simulink model "ConSys_A1"  (Simulink 8.3)
settings: Solver=ode3  StartTime=0.0  StopTime=Time(end)  FixedStep=Ts  RelTol=1e-3
values from neighbouring files (symbols this model uses):
  d = r*h    (= 1.6)    [StartUp_A1.m]
  d0 = d*h    (= 0.0032)    [StartUp_A1.m]
  h = 0.002    [StartUp_A1.m]
  Ka = diag([ 3  20  20  150  355  520])    [StartUp_A1.m]
  Kd = diag([ 3   5  25  100   15 1050])    [StartUp_A1.m]
  Ki = diag([35 555 810 7410 1850 5815])    [StartUp_A1.m]
  Kp = diag([55 180 350 1960  680 4450])    [StartUp_A1.m]
  r = 800    [StartUp_A1.m]
  TD = ss(Atd,Btd,Ctd,Dtd,Ts)    [StartUp_A1.m]
  Ts = 1/200    (= 0.005)    [StartUp_A1.m]
undefined symbols (not defined in the file or in its folder): DiscIntNeverNeededParam
undefined symbols (not defined in the file): ADAMS_cwd, ADAMS_exec, ADAMS_host, ADAMS_init, ADAMS_inputs, ADAMS_outputs, ADAMS_prefix, ADAMS_static, ADAMS_sysdir
libraries: cstblocks x6
(part 7 of 9)

== matlab function A2/MATLAB Function 4 ==
  data: q input double; V4 output double; dq input double
function V4 = V4(q,dq)
%#codegen
Th1=q(1,1); Th2=q(2,1); Th3=q(3,1); Th4=q(4,1); Th5=q(5,1); Th6=q(6,1);
dTh1=dq(1); dTh2=dq(2); dTh3=dq(3); dTh4=dq(4); dTh5=dq(5); dTh6=dq(6);
%---------------------------
V411=((0.000115*cos(Th4)*sin(Th6) - 0.02603*sin(Th4)*sin(Th5) + 0.000115*cos(Th5)*cos(Th6)*sin(Th4))*(0.07*sin(Th2 + Th3) + 0.063*sin(2.0*Th2 + 2.0*Th3) - 0.36*sin(Th2 + Th3)*sin(Th2) + 0.05206*cos(Th4)*sin(Th5) + 0.00023*sin(Th4)*sin(Th6) + 0.254*sin(Th2 + Th3)*cos(Th2)*cos(Th3) - 0.254*sin(Th2 + Th3)*sin(Th2)*sin(Th3) - 0.00023*cos(Th4)*cos(Th5)*cos(Th6) - 0.05206*sin(Th2 + Th3)^2*cos(Th4)*sin(Th5) - 0.00023*sin(Th2 + Th3)^2*sin(Th4)*sin(Th6) + 0.05206*cos(Th2 + Th3)*sin(Th2 + Th3)*cos(Th5) + 0.00023*sin(Th2 + Th3)^2*cos(Th4)*cos(Th5)*cos(Th6) + 0.00023*cos(Th2 + Th3)*sin(Th2 + Th3)*cos(Th6)*sin(Th5)) - 1.0*(0.00062*cos(Th4) - 0.00002*cos(Th5)*sin(Th4) + 0.00152*sin(Th4)*sin(Th5))*(0.00062*sin(Th2 + Th3)^2*sin(Th4) - 0.063*sin(2.0*Th2 + 2.0*Th3) - 0.00062*sin(Th4) - 0.07*sin(Th2 + Th3) + 0.36*sin(Th2 + Th3)*sin(Th2) - 0.00002*cos(Th4)*cos(Th5) + 0.00152*cos(Th4)*sin(Th5) + 0.00002*cos(Th2 + Th3)*sin(Th2 + Th3)*sin(Th5) - 0.254*sin(Th2 + Th3)*cos(Th2)*cos(Th3) + 0.254*sin(Th2 + Th3)*sin(Th2)*sin(Th3) + 0.00002*sin(Th2 + Th3)^2*cos(Th4)*cos(Th5) - 0.00152*sin(Th2 + Th3)^2*cos(Th4)*sin(Th5) + 0.00152*cos(Th2 + Th3)*sin(Th2 + Th3)*cos(Th5)) - 1.1369e-18*cos(Th2 + Th3)*(3.5184e13*cos(Th2 + Th3)*sin(Th5) + 4.1368e15*cos(Th2 + Th3)*cos(Th4)*sin(Th4) - 3.5184e13*sin(Th2 + Th3)*cos(Th4)*cos(Th5) - 7.0369e13*cos(Th2 + Th3)*cos(Th4)^2*sin(Th5) + 3.8782e15*sin(Th2 + Th3)*cos(Th5)*sin(Th4)*sin(Th5) - 3.8782e15*cos(Th2 + Th3)*cos(Th4)*cos(Th5)^2*sin(Th4)) - 4.2352e-22*cos(Th2 + Th3)*(1.2314e18*cos(Th4)*sin(Th6) + 4.7224e15*sin(Th4)*sin(Th5) + 1.2314e18*cos(Th5)*cos(Th6)*sin(Th4))*(cos(Th2 + Th3)*sin(Th4)*sin(Th6) + sin(Th2 + Th3)*cos(Th6)*sin(Th5) - 1.0*cos(Th2 + Th3)*cos(Th4)*cos(Th5)*cos(Th6)) - 0.00052*cos(Th2 + Th3)*(cos(Th4)*cos(Th6) - 1.0*cos(Th5)*sin(Th4)*sin(Th6))*(cos(Th2 + Th3)*cos(Th6)*sin(Th4) - 1.0*sin(Th2 + Th3)*sin(Th5)*sin(Th6) + cos(Th2 + Th3)*cos(Th4)*cos(Th5)*sin(Th6)) - 0.004593*cos(Th2 + Th3)^2*cos(Th4)*sin(Th4) - 0.5*cos(Th2 + Th3)*(cos(Th4)*cos(Th6) - 1.0*cos(Th5)*sin(Th4)*sin(Th6))*(0.00104*cos(Th2 + Th3)*cos(Th6)*sin(Th4) - 0.00104*sin(Th2 + Th3)*sin(Th5)*sin(Th6) + 0.00104*cos(Th2 + Th3)*cos(Th4)*cos(Th5)*sin(Th6)) + 0.5*cos(Th2 + Th3)*(cos(Th4)*sin(Th6) + cos(Th5)*cos(Th6)*sin(Th4))*(4.0e-6*sin(Th2 + Th3)*cos(Th5) + 4.0e-6*cos(Th2 + Th3)*cos(Th4)*sin(Th5) - 0.001043*cos(Th2 + Th3)*sin(Th4)*sin(Th6) - 0.001043*sin(Th2 + Th3)*cos(Th6)*sin(Th5) + 0.001043*cos(Th2 + Th3)*cos(Th4)*cos(Th5)*cos(Th6)) + 4.2352e-22*cos(Th2 + Th3)*(sin(Th2 + Th3)*cos(Th5) + cos(Th2 + Th3)*cos(Th4)*sin(Th5))*(4.7224e15*cos(Th4)*sin(Th6) + 1.3695e17*sin(Th4)*sin(Th5) + 4.7224e15*cos(Th5)*cos(Th6)*sin(Th4)) + 0.5*cos(Th2 + Th3)*sin(Th4)*sin(Th5)*(0.000116*sin(Th2 + Th3)*cos(Th5) + 0.000116*cos(Th2 + Th3)*cos(Th4)*sin(Th5) - 4.0e-6*cos(Th2 + Th3)*sin(Th4)*sin(Th6) - 4.0e-6*sin(Th2 + Th3)*cos(Th6)*sin(Th5) + 4.0e-6*cos(Th2 + Th3)*cos(Th4)*cos(Th5)*cos(Th6)))*dTh1*dTh1;
V412=(0.0064488*cos(Th2)*cos(Th3) + 0.0003348*cos(Th2)*sin(Th4) - 0.0064488*sin(Th2)*sin(Th3) - 0.01158*cos(Th4)^2*sin(Th2)*sin(Th3) + 0.0033452*cos(Th5)^2*sin(Th2)*sin(Th3) - 4.4603e-6*cos(Th6)^2*sin(Th2)*sin(Th3) + 0.0000108*cos(Th2)*cos(Th4)*cos(Th5) + 4.56e-8*cos(Th2)*cos(Th4)*sin(Th3) + 4.56e-8*cos(Th3)*cos(Th4)*sin(Th2) + 0.013235*cos(Th2)*cos(Th4)*sin(Th5) + 0.0003534*cos(Th2)*sin(Th3)*sin(Th4) + 0.0003534*cos(Th3)*sin(Th2)*sin(Th4) + 0.0000621*cos(Th2)*sin(Th4)*sin(Th6) + 0.01158*cos(Th2)*cos(Th3)*cos(Th4)^2 - 0.0033452*cos(Th2)*cos(Th3)*cos(Th5)^2 + 4.4603e-6*cos(Th2)*cos(Th3)*cos(Th6)^2 + 0.0066904*cos(Th4)^2*cos(Th5)^2*sin(Th2)*sin(Th3) + 2.9736e-6*cos(Th4)^2*cos(Th6)^2*sin(Th2)*sin(Th3) + 1.4868e-6*cos(Th5)^2*cos(Th6)^2*sin(Th2)*sin(Th3) - 0.0000621*cos(Th2)*cos(Th4)*cos(Th5)*cos(Th6) + 0.0000114*cos(Th2)*cos(Th4)*cos(Th5)*sin(Th3) + 0.0000114*cos(Th3)*cos(Th4)*cos(Th5)*sin(Th2) - 3.04e-8*cos(Th2)*cos(Th3)*cos(Th5)*sin(Th5) + 0.00001498*cos(Th2)*cos(Th4)*cos(Th6)*sin(Th3) + 0.00001498*cos(Th3)*cos(Th4)*cos(Th6)*sin(Th2) + 0.013971*cos(Th2)*cos(Th4)*sin(Th3)*sin(Th5) + 0.000058586*cos(Th2)*cos(Th5)*sin(Th3)*sin(Th4) + 0.013971*cos(Th3)*cos(Th4)*sin(Th2)*sin(Th5) + 0.000058586*cos(Th3)*cos(Th5)*sin(Th2)*sin(Th4) - 1.86e-8*cos(Th2)*sin(Th3)*sin(Th4)*sin(Th5) - 1.86e-8*cos(Th3)*sin(Th2)*sin(Th4)*sin(Th5) + 0.00006555*cos(Th2)*sin(Th3)*sin(Th4)*sin(Th6) + 0.00006555*cos(Th3)*sin(Th2)*sin(Th4)*sin(Th6) + 3.04e-8*cos(Th5)*sin(Th2)*sin(Th3)*sin(Th5) - 9.12e-8*cos(Th2)*cos(Th4)*cos(Th5)^2*sin(Th3) - 9.12e-8*cos(Th3)*cos(Th4)*cos(Th5)^2*sin(Th2) - 0.0066904*cos(Th2)*cos(Th3)*cos(Th4)^2*cos(Th5)^2 - 2.9736e-6*cos(Th2)*cos(Th3)*cos(Th4)^2*cos(Th6)^2 - 1.4868e-6*cos(Th2)*cos(Th3)*cos(Th5)^2*cos(Th6)^2 + 2.48e-8*cos(Th2)*cos(Th3)*cos(Th4)*cos(Th5)*sin(Th4) - 0.00006555*cos(Th2)*cos(Th4)*cos(Th5)*cos(Th6)*sin(Th3) - 0.00006555*cos(Th3)*cos(Th4)*cos(Th5)*cos(Th6)*sin(Th2) - 9.9869e-6*cos(Th2)*cos(Th3)*cos(Th5)*cos(Th6)*sin(Th5) - 2.9736e-6*cos(Th2)*cos(Th3)*cos(Th4)^2*cos(Th5)^2*cos(Th6)^2 + 0.000078115*cos(Th2)*cos(Th3)*cos(Th4)*sin(Th4)*sin(Th5) + 0.010036*cos(Th2)*cos(Th4)*cos(Th5)*sin(Th3)*sin(Th5) + 0.010036*cos(Th3)*cos(Th4)*cos(Th5)*sin(Th2)*sin(Th5) - 2.48e-8*cos(Th4)*cos(Th5)*sin(Th2)*sin(Th3)*sin(Th4) + 0.00001498*cos(Th2)*cos(Th5)*sin(Th3)*sin(Th4)*sin(Th6) + 0.00001498*cos(Th3)*cos(Th5)*sin(Th2)*sin(Th4)*sin(Th6) + 9.9869e-6*cos(Th5)*cos(Th6)*sin(Th2)*sin(Th3)*sin(Th5) + 2.9736e-6*cos(Th4)^2*cos(Th5)^2*cos(Th6)^2*sin(Th2)*sin(Th3) - 0.000078115*cos(Th4)*sin(Th2)*sin(Th3)*sin(Th4)*sin(Th5) - 6.08e-8*cos(Th2)*cos(Th3)*cos(Th4)^2*cos(Th5)*sin(Th5) - 0.000029961*cos(Th2)*cos(Th4)*cos(Th5)^2*cos(Th6)*sin(Th3) - 0.000029961*cos(Th3)*cos(Th4)*cos(Th5)^2*cos(Th6)*sin(Th2) + 6.08e-8*cos(Th4)^2*cos(Th5)*sin(Th2)*sin(Th3)*sin(Th5) - 0.000019974*cos(Th2)*cos(Th3)*cos(Th4)^2*cos(Th5)*cos(Th6)*sin(Th5) + 4.4603e-6*cos(Th2)*cos(Th4)*cos(Th5)*cos(Th6)^2*sin(Th3)*sin(Th5) + 4.4603e-6*cos(Th3)*cos(Th4)*cos(Th5)*cos(Th6)^2*sin(Th2)*sin(Th5) + 0.000019974*cos(Th4)^2*cos(Th5)*cos(Th6)*sin(Th2)*sin(Th3)*sin(Th5) + 0.000019974*cos(Th2)*cos(Th3)*cos(Th4)*sin(Th4)*sin(Th5)*sin(Th6) - 4.4603e-6*cos(Th2)*cos(Th6)*sin(Th3)*sin(Th4)*sin(Th5)*sin(Th6) - 4.4603e-6*cos(Th3)*cos(Th6)*sin(Th2)*sin(Th4)*sin(Th5)*sin(Th6) - 0.000019974*cos(Th4)*sin(Th2)*sin(Th3)*sin(Th4)*sin(Th5)*sin(Th6) + 5.9471e-6*cos(Th2)*cos(Th3)*cos(Th4)*cos(Th5)*cos(Th6)*sin(Th4)*sin(Th6) - 5.9471e-6*cos(Th4)*cos(Th5)*cos(Th6)*sin(Th2)*sin(Th3)*sin(Th4)*sin(Th6))*dTh1*dTh2;
V413=(0.0064488*cos(Th2)*cos(Th3) - 0.0064488*sin(Th2)*sin(Th3) - 0.01158*cos(Th4)^2*sin(Th2)*sin(Th3) + 0.0033452*cos(Th5)^2*sin(Th2)*sin(Th3) - 4.4603e-6*cos(Th6)^2*sin(Th2)*sin(Th3) + 4.56e-8*cos(Th2)*cos(Th4)*sin(Th3) + 4.56e-8*cos(Th3)*cos(Th4)*sin(Th2) + 0.0003534*cos(Th2)*sin(Th3)*sin(Th4) + 0.0003534*cos(Th3)*sin(Th2)*sin(Th4) + 0.01158*cos(Th2)*cos(Th3)*cos(Th4)^2 - 0.0033452*cos(Th2)*cos(Th3)*cos(Th5)^2 + 4.4603e-6*cos(Th2)*cos(Th3)*cos(Th6)^2 + 0.0066904*cos(Th4)^2*cos(Th5)^2*sin(Th2)*sin(Th3) + 2.9736e-6*cos(Th4)^2*cos(Th6)^2*sin(Th2)*sin(Th3) + 1.4868e-6*cos(Th5)^2*cos(Th6)^2*sin(Th2)*sin(Th3) + 0.0000114*cos(Th2)*cos(Th4)*cos(Th5)*sin(Th3) + 0.0000114*cos(Th3)*cos(Th4)*cos(Th5)*sin(Th2) - 3.04e-8*cos(Th2)*cos(Th3)*cos(Th5)*sin(Th5) + 0.00001498*cos(Th2)*cos(Th4)*cos(Th6)*sin(Th3) + 0.00001498*cos(Th3)*cos(Th4)*cos(Th6)*sin(Th2) + 0.013971*cos(Th2)*cos(Th4)*sin(Th3)*sin(Th5) + 0.000058586*cos(Th2)*cos(Th5)*sin(Th3)*sin(Th4) + 0.013971*cos(Th3)*cos(Th4)*sin(Th2)*sin(Th5) + 0.000058586*cos(Th3)*cos(Th5)*sin(Th2)*sin(Th4) - 1.86e-8*cos(Th2)*sin(Th3)*sin(Th4)*sin(Th5) - 1.86e-8*cos(Th3)*sin(Th2)*sin(Th4)*sin(Th5) + 0.00006555*cos(Th2)*sin(Th3)*sin(Th4)*sin(Th6) + 0.00006555*cos(Th3)*sin(Th2)*sin(Th4)*sin(Th6) + 3.04e-8*cos(Th5)*sin(Th2)*sin(Th3)*sin(Th5) - 9.12e-8*cos(Th2)*cos(Th4)*cos(Th5)^2*sin(Th3) - 9.12e-8*cos(Th3)*cos(Th4)*cos(Th5)^2*sin(Th2) - 0.0066904*cos(Th2)*cos(Th3)*cos(Th4)^2*cos(Th5)^2 - 2.9736e-6*cos(Th2)*cos(Th3)*cos(Th4)^2*cos(Th6)^2 - 1.4868e-6*cos(Th2)*cos(Th3)*cos(Th5)^2*cos(Th6)^2 + 2.48e-8*cos(Th2)*cos(Th3)*cos(Th4)*cos(Th5)*sin(Th4) - 0.00006555*cos(Th2)*cos(Th4)*cos(Th5)*cos(Th6)*sin(Th3) - 0.00006555*cos(Th3)*cos(Th4)*cos(Th5)*cos(Th6)*sin(Th2) - 9.9869e-6*cos(Th2)*cos(Th3)*cos(Th5)*cos(Th6)*sin(Th5) - 2.9736e-6*cos(Th2)*cos(Th3)*cos(Th4)^2*cos(Th5)^2*cos(Th6)^2 + 0.000078115*cos(Th2)*cos(Th3)*cos(Th4)*sin(Th4)*sin(Th5) + 0.010036*cos(Th2)*cos(Th4)*cos(Th5)*sin(Th3)*sin(Th5) + 0.010036*cos(Th3)*cos(Th4)*cos(Th5)*sin(Th2)*sin(Th5) - 2.48e-8*cos(Th4)*cos(Th5)*sin(Th2)*sin(Th3)*sin(Th4) + 0.00001498*cos(Th2)*cos(Th5)*sin(Th3)*sin(Th4)*sin(Th6) + 0.00001498*cos(Th3)*cos(Th5)*sin(Th2)*sin(Th4)*sin(Th6) + 9.9869e-6*cos(Th5)*cos(Th6)*sin(Th2)*sin(Th3)*sin(Th5) + 2.9736e-6*cos(Th4)^2*cos(Th5)^2*cos(Th6)^2*sin(Th2)*sin(Th3) - 0.000078115*cos(Th4)*sin(Th2)*sin(Th3)*sin(Th4)*sin(Th5) - 6.08e-8*cos(Th2)*cos(Th3)*cos(Th4)^2*cos(Th5)*sin(Th5) - 0.000029961*cos(Th2)*cos(Th4)*cos(Th5)^2*cos(Th6)*sin(Th3) - 0.000029961*cos(Th3)*cos(Th4)*cos(Th5)^2*cos(Th6)*sin(Th2) + 6.08e-8*cos(Th4)^2*cos(Th5)*sin(Th2)*sin(Th3)*sin(Th5) - 0.000019974*cos(Th2)*cos(Th3)*cos(Th4)^2*cos(Th5)*cos(Th6)*sin(Th5) + 4.4603e-6*cos(Th2)*cos(Th4)*cos(Th5)*cos(Th6)^2*sin(Th3)*sin(Th5) + 4.4603e-6*cos(Th3)*cos(Th4)*cos(Th5)*cos(Th6)^2*sin(Th2)*sin(Th5) + 0.000019974*cos(Th4)^2*cos(Th5)*cos(Th6)*sin(Th2)*sin(Th3)*sin(Th5) + 0.000019974*cos(Th2)*cos(Th3)*cos(Th4)*sin(Th4)*sin(Th5)*sin(Th6) - 4.4603e-6*cos(Th2)*cos(Th6)*sin(Th3)*sin(Th4)*sin(Th5)*sin(Th6) - 4.4603e-6*cos(Th3)*cos(Th6)*sin(Th2)*sin(Th4)*sin(Th5)*sin(Th6) - 0.000019974*cos(Th4)*sin(Th2)*sin(Th3)*sin(Th4)*sin(Th5)*sin(Th6) + 5.9471e-6*cos(Th2)*cos(Th3)*cos(Th4)*cos(Th5)*cos(Th6)*sin(Th4)*sin(Th6) - 5.9471e-6*cos(Th4)*cos(Th5)*cos(Th6)*sin(Th2)*sin(Th3)*sin(Th4)*sin(Th6))*dTh1*dTh3;
V414=(0.0001116*cos(Th4)*sin(Th2) - 0.0000217*cos(Th4) + 7.0e-7*cos(Th5)*sin(Th4) - 4.025e-6*cos(Th4)*sin(Th6) + 0.00085785*sin(Th4)*sin(Th5) - 0.0001178*cos(Th2)*cos(Th3)*cos(Th4) + 1.52e-8*cos(Th2)*cos(Th3)*sin(Th4) - 4.025e-6*cos(Th5)*cos(Th6)*sin(Th4) + 0.0001178*cos(Th4)*sin(Th2)*sin(Th3) - 3.6e-6*cos(Th5)*sin(Th2)*sin(Th4) + 0.0000207*cos(Th4)*sin(Th2)*sin(Th6) - 1.52e-8*sin(Th2)*sin(Th3)*sin(Th4) - 0.0044118*sin(Th2)*sin(Th4)*sin(Th5) - 0.000019529*cos(Th2)*cos(Th3)*cos(Th4)*cos(Th5) + 6.2e-9*cos(Th2)*cos(Th3)*cos(Th4)*sin(Th5) + 3.8e-6*cos(Th2)*cos(Th3)*cos(Th5)*sin(Th4) - 0.00002185*cos(Th2)*cos(Th3)*cos(Th4)*sin(Th6) + 4.9934e-6*cos(Th2)*cos(Th3)*cos(Th6)*sin(Th4) + 0.0046569*cos(Th2)*cos(Th3)*sin(Th4)*sin(Th5) + 0.000019529*cos(Th4)*cos(Th5)*sin(Th2)*sin(Th3) + 0.0000207*cos(Th5)*cos(Th6)*sin(Th2)*sin(Th4) - 6.2e-9*cos(Th4)*sin(Th2)*sin(Th3)*sin(Th5) - 3.8e-6*cos(Th5)*sin(Th2)*sin(Th3)*sin(Th4) + 0.00002185*cos(Th4)*sin(Th2)*sin(Th3)*sin(Th6) - 4.9934e-6*cos(Th6)*sin(Th2)*sin(Th3)*sin(Th4) - 0.0046569*sin(Th2)*sin(Th3)*sin(Th4)*sin(Th5) - 3.04e-8*cos(Th2)*cos(Th3)*cos(Th5)^2*sin(Th4) + 3.04e-8*cos(Th5)^2*sin(Th2)*sin(Th3)*sin(Th4) - 4.9934e-6*cos(Th2)*cos(Th3)*cos(Th4)*cos(Th5)*sin(Th6) - 0.00002185*cos(Th2)*cos(Th3)*cos(Th5)*cos(Th6)*sin(Th4) + 0.0033452*cos(Th2)*cos(Th3)*cos(Th5)*sin(Th4)*sin(Th5) + 4.9934e-6*cos(Th4)*cos(Th5)*sin(Th2)*sin(Th3)*sin(Th6) + 0.00002185*cos(Th5)*cos(Th6)*sin(Th2)*sin(Th3)*sin(Th4) - 0.0033452*cos(Th5)*sin(Th2)*sin(Th3)*sin(Th4)*sin(Th5) - 9.9869e-6*cos(Th2)*cos(Th3)*cos(Th5)^2*cos(Th6)*sin(Th4) + 9.9869e-6*cos(Th5)^2*cos(Th6)*sin(Th2)*sin(Th3)*sin(Th4) + 1.4868e-6*cos(Th2)*cos(Th3)*cos(Th5)*cos(Th6)^2*sin(Th4)*sin(Th5) - 1.4868e-6*cos(Th5)*cos(Th6)^2*sin(Th2)*sin(Th3)*sin(Th4)*sin(Th5) + 1.4868e-6*cos(Th2)*cos(Th3)*cos(Th4)*cos(Th6)*sin(Th5)*sin(Th6) - 1.4868e-6*cos(Th4)*cos(Th6)*sin(Th2)*sin(Th3)*sin(Th5)*sin(Th6))*dTh1*dTh4;
V415=(6.08e-8*cos(Th2)*sin(Th3) - 0.00085785*cos(Th4)*cos(Th5) + 6.08e-8*cos(Th3)*sin(Th2) + 7.0e-7*cos(Th4)*sin(Th5) + 0.010487*cos(Th2)*cos(Th3)*cos(Th4) + 0.000019974*cos(Th2)*cos(Th6)*sin(Th3) + 0.000019974*cos(Th3)*cos(Th6)*sin(Th2) + 0.0044118*cos(Th4)*cos(Th5)*sin(Th2) - 4.025e-6*cos(Th4)*cos(Th6)*sin(Th5) - 0.010487*cos(Th4)*sin(Th2)*sin(Th3) - 3.6e-6*cos(Th4)*sin(Th2)*sin(Th5) - 1.216e-7*cos(Th2)*cos(Th5)^2*sin(Th3) - 1.216e-7*cos(Th3)*cos(Th5)^2*sin(Th2) - 0.0046569*cos(Th2)*cos(Th3)*cos(Th4)*cos(Th5) + 3.8e-6*cos(Th2)*cos(Th3)*cos(Th4)*sin(Th5) + 1.86e-8*cos(Th2)*cos(Th3)*cos(Th5)*sin(Th4) + 0.000058586*cos(Th2)*cos(Th3)*sin(Th4)*sin(Th5) + 0.0046569*cos(Th4)*cos(Th5)*sin(Th2)*sin(Th3) + 0.013381*cos(Th2)*cos(Th5)*sin(Th3)*sin(Th5) + 0.013381*cos(Th3)*cos(Th5)*sin(Th2)*sin(Th5) + 0.0000207*cos(Th4)*cos(Th6)*sin(Th2)*sin(Th5) - 3.8e-6*cos(Th4)*sin(Th2)*sin(Th3)*sin(Th5) - 1.86e-8*cos(Th5)*sin(Th2)*sin(Th3)*sin(Th4) - 0.000058586*sin(Th2)*sin(Th3)*sin(Th4)*sin(Th5) - 0.013381*cos(Th2)*cos(Th3)*cos(Th4)*cos(Th5)^2 + 1.4868e-6*cos(Th2)*cos(Th3)*cos(Th4)*cos(Th6)^2 - 0.000039948*cos(Th2)*cos(Th5)^2*cos(Th6)*sin(Th3) - 0.000039948*cos(Th3)*cos(Th5)^2*cos(Th6)*sin(Th2) + 0.013381*cos(Th4)*cos(Th5)^2*sin(Th2)*sin(Th3) - 1.4868e-6*cos(Th4)*cos(Th6)^2*sin(Th2)*sin(Th3) - 1.216e-7*cos(Th2)*cos(Th3)*cos(Th4)*cos(Th5)*sin(Th5) - 0.00002185*cos(Th2)*cos(Th3)*cos(Th4)*cos(Th6)*sin(Th5) + 1.216e-7*cos(Th4)*cos(Th5)*sin(Th2)*sin(Th3)*sin(Th5) + 0.00001498*cos(Th2)*cos(Th3)*sin(Th4)*sin(Th5)*sin(Th6) + 0.00002185*cos(Th4)*cos(Th6)*sin(Th2)*sin(Th3)*sin(Th5) - 0.00001498*sin(Th2)*sin(Th3)*sin(Th4)*sin(Th5)*sin(Th6) + 5.9471e-6*cos(Th2)*cos(Th5)*cos(Th6)^2*sin(Th3)*sin(Th5) + 5.9471e-6*cos(Th3)*cos(Th5)*cos(Th6)^2*sin(Th2)*sin(Th5) - 5.9471e-6*cos(Th2)*cos(Th3)*cos(Th4)*cos(Th5)^2*cos(Th6)^2 + 5.9471e-6*cos(Th4)*cos(Th5)^2*cos(Th6)^2*sin(Th2)*sin(Th3) - 0.000039948*cos(Th2)*cos(Th3)*cos(Th4)*cos(Th5)*cos(Th6)*sin(Th5) + 4.4603e-6*cos(Th2)*cos(Th3)*cos(Th5)*cos(Th6)*sin(Th4)*sin(Th6) + 0.000039948*cos(Th4)*cos(Th5)*cos(Th6)*sin(Th2)*sin(Th3)*sin(Th5) - 4.4603e-6*cos(Th5)*cos(Th6)*sin(Th2)*sin(Th3)*sin(Th4)*sin(Th6))*dTh1*dTh5;
V416=(0.0000207*cos(Th6)*sin(Th2)*sin(Th4) - 4.025e-6*cos(Th4)*cos(Th5)*sin(Th6) - 4.025e-6*cos(Th6)*sin(Th4) + 0.00001498*cos(Th2)*cos(Th3)*cos(Th4)*sin(Th6) - 0.00002185*cos(Th2)*cos(Th3)*cos(Th6)*sin(Th4) + 0.00005504*cos(Th2)*cos(Th3)*sin(Th4)*sin(Th5) - 5.9471e-6*cos(Th2)*cos(Th6)*sin(Th3)*sin(Th6) - 5.9471e-6*cos(Th3)*cos(Th6)*sin(Th2)*sin(Th6) + 0.0000207*cos(Th4)*cos(Th5)*sin(Th2)*sin(Th6) - 0.00001498*cos(Th4)*sin(Th2)*sin(Th3)*sin(Th6) + 0.00002185*cos(Th6)*sin(Th2)*sin(Th3)*sin(Th4) - 0.00005504*sin(Th2)*sin(Th3)*sin(Th4)*sin(Th5) - 0.00002185*cos(Th2)*cos(Th3)*cos(Th4)*cos(Th5)*sin(Th6) - 4.9934e-6*cos(Th2)*cos(Th3)*cos(Th5)*cos(Th6)*sin(Th4) + 0.00002185*cos(Th4)*cos(Th5)*sin(Th2)*sin(Th3)*sin(Th6) + 4.9934e-6*cos(Th5)*cos(Th6)*sin(Th2)*sin(Th3)*sin(Th4) + 0.000019974*cos(Th2)*cos(Th5)*sin(Th3)*sin(Th5)*sin(Th6) + 0.000019974*cos(Th3)*cos(Th5)*sin(Th2)*sin(Th5)*sin(Th6) - 0.000019974*cos(Th2)*cos(Th3)*cos(Th4)*cos(Th5)^2*sin(Th6) + 5.9471e-6*cos(Th2)*cos(Th3)*cos(Th6)^2*sin(Th4)*sin(Th5) + 5.9471e-6*cos(Th2)*cos(Th5)^2*cos(Th6)*sin(Th3)*sin(Th6) + 5.9471e-6*cos(Th3)*cos(Th5)^2*cos(Th6)*sin(Th2)*sin(Th6) + 0.000019974*cos(Th4)*cos(Th5)^2*sin(Th2)*sin(Th3)*sin(Th6) - 5.9471e-6*cos(Th6)^2*sin(Th2)*sin(Th3)*sin(Th4)*sin(Th5) + 5.9471e-6*cos(Th2)*cos(Th3)*cos(Th4)*cos(Th5)*cos(Th6)*sin(Th5)*sin(Th6) - 5.9471e-6*cos(Th4)*cos(Th5)*cos(Th6)*sin(Th2)*sin(Th3)*sin(Th5)*sin(Th6))*dTh1*dTh6;
%---------------------------
V421=(0.5*(0.02603*cos(Th4)*sin(Th5) + 0.000115*sin(Th4)*sin(Th6) - 0.000115*cos(Th4)*cos(Th5)*cos(Th6))*(0.126*sin(Th2 + Th3) + 0.36*cos(Th2) + 0.05206*sin(Th2 + Th3)*cos(Th5) + 0.254*cos(Th2)*sin(Th3) + 0.254*cos(Th3)*sin(Th2) + 0.05206*cos(Th2 + Th3)*cos(Th4)*sin(Th5) + 0.00023*cos(Th2 + Th3)*sin(Th4)*sin(Th6) + 0.00023*sin(Th2 + Th3)*cos(Th6)*sin(Th5) - 0.00023*cos(Th2 + Th3)*cos(Th4)*cos(Th5)*cos(Th6)) - 2.5e-11*cos(Th2 + Th3)*(23.0*cos(Th4)*sin(Th6) - 5206.0*sin(Th4)*sin(Th5) + 23.0*cos(Th5)*cos(Th6)*sin(Th4))^2 - 0.0051115*cos(Th2 + Th3) + 0.5*(0.00062*sin(Th4) + 0.00002*cos(Th4)*cos(Th5) - 0.00152*cos(Th4)*sin(Th5))*(0.126*sin(Th2 + Th3) + 0.36*cos(Th2) + 0.00062*cos(Th2 + Th3)*sin(Th4) - 0.00152*sin(Th2 + Th3)*cos(Th5) - 0.00002*sin(Th2 + Th3)*sin(Th5) + 0.254*cos(Th2)*sin(Th3) + 0.254*cos(Th3)*sin(Th2) + 0.00002*cos(Th2 + Th3)*cos(Th4)*cos(Th5) - 0.00152*cos(Th2 + Th3)*cos(Th4)*sin(Th5)) + 0.010223*cos(Th2 + Th3)*cos(Th4)^2 + 0.0026665*cos(Th2 + Th3)*cos(Th5)^2 + 1.5e-6*cos(Th2 + Th3)*cos(Th6)^2 - 2.0e-10*cos(Th2 + Th3)*(31.0*cos(Th4) - 1.0*cos(Th5)*sin(Th4) + 76.0*sin(Th4)*sin(Th5))^2 + 2.0e-6*sin(Th2 + Th3)*cos(Th4)*cos(Th6) + 0.00002*sin(Th2 + Th3)*cos(Th5)*sin(Th4) - 0.005333*cos(Th2 + Th3)*cos(Th4)^2*cos(Th5)^2 - 3.0e-6*cos(Th2 + Th3)*cos(Th4)^2*cos(Th6)^2 + 1.5e-6*cos(Th2 + Th3)*cos(Th5)^2*cos(Th6)^2 + 4.0e-6*cos(Th2 + Th3)*cos(Th5)*cos(Th6)*sin(Th5) - 3.0e-6*cos(Th2 + Th3)*cos(Th4)^2*cos(Th5)^2*cos(Th6)^2 + 0.00008*cos(Th2 + Th3)*cos(Th4)*sin(Th4)*sin(Th5) + 0.0026665*sin(Th2 + Th3)*cos(Th4)*cos(Th5)*sin(Th5) + 2.0e-6*sin(Th2 + Th3)*cos(Th5)*sin(Th4)*sin(Th6) - 4.0e-6*sin(Th2 + Th3)*cos(Th4)*cos(Th5)^2*cos(Th6) - 8.0e-6*cos(Th2 + Th3)*cos(Th4)^2*cos(Th5)*cos(Th6)*sin(Th5) + 1.5e-6*sin(Th2 + Th3)*cos(Th4)*cos(Th5)*cos(Th6)^2*sin(Th5) + 8.0e-6*cos(Th2 + Th3)*cos(Th4)*sin(Th4)*sin(Th5)*sin(Th6) - 1.5e-6*sin(Th2 + Th3)*cos(Th6)*sin(Th4)*sin(Th5)*sin(Th6) + 6.0e-6*cos(Th2 + Th3)*cos(Th4)*cos(Th5)*cos(Th6)*sin(Th4)*sin(Th6))*dTh2*dTh1;
V422=(0.00579*sin(2.0*Th4) + 1.24e-8*cos(Th5) + 0.000039058*sin(Th5) - 2.48e-8*cos(Th4)^2*cos(Th5) - 0.000078115*cos(Th4)^2*sin(Th5) - 0.0002232*cos(Th3)*cos(Th4) + 9.9869e-6*sin(Th5)*sin(Th6) - 0.000019974*cos(Th4)^2*sin(Th5)*sin(Th6) + 7.2e-6*cos(Th3)*cos(Th5)*sin(Th4) - 0.0000414*cos(Th3)*cos(Th4)*sin(Th6) + 2.9736e-6*cos(Th5)*cos(Th6)*sin(Th6) + 0.0088236*cos(Th3)*sin(Th4)*sin(Th5) - 0.0066904*cos(Th4)*cos(Th5)^2*sin(Th4) - 2.9736e-6*cos(Th4)*cos(Th6)^2*sin(Th4) - 2.9736e-6*cos(Th4)*cos(Th5)^2*cos(Th6)^2*sin(Th4) - 0.0000414*cos(Th3)*cos(Th5)*cos(Th6)*sin(Th4) - 6.08e-8*cos(Th4)*cos(Th5)*sin(Th4)*sin(Th5) - 5.9471e-6*cos(Th4)^2*cos(Th5)*cos(Th6)*sin(Th6) - 0.000019974*cos(Th4)*cos(Th5)*cos(Th6)*sin(Th4)*sin(Th5))*dTh2*dTh2;
V423=(0.00579*sin(2.0*Th4) + 1.24e-8*cos(Th5) + 0.000039058*sin(Th5) - 2.48e-8*cos(Th4)^2*cos(Th5) - 0.000078115*cos(Th4)^2*sin(Th5) + 0.0001116*cos(Th3)*cos(Th4) + 9.9869e-6*sin(Th5)*sin(Th6) - 0.000019974*cos(Th4)^2*sin(Th5)*sin(Th6) - 3.6e-6*cos(Th3)*cos(Th5)*sin(Th4) + 0.0000207*cos(Th3)*cos(Th4)*sin(Th6) + 2.9736e-6*cos(Th5)*cos(Th6)*sin(Th6) - 0.0044118*cos(Th3)*sin(Th4)*sin(Th5) - 0.0066904*cos(Th4)*cos(Th5)^2*sin(Th4) - 2.9736e-6*cos(Th4)*cos(Th6)^2*sin(Th4) - 2.9736e-6*cos(Th4)*cos(Th5)^2*cos(Th6)^2*sin(Th4) + 0.0000207*cos(Th3)*cos(Th5)*cos(Th6)*sin(Th4) - 6.08e-8*cos(Th4)*cos(Th5)*sin(Th4)*sin(Th5) - 5.9471e-6*cos(Th4)^2*cos(Th5)*cos(Th6)*sin(Th6) - 0.000019974*cos(Th4)*cos(Th5)*cos(Th6)*sin(Th4)*sin(Th5))*dTh2*dTh3;
V424=(3.04e-8*cos(Th4)*cos(Th5)^2 - 0.0001178*sin(Th4) - 1.52e-8*cos(Th4) - 3.8e-6*cos(Th4)*cos(Th5) - 4.9934e-6*cos(Th4)*cos(Th6) - 0.0046569*cos(Th4)*sin(Th5) - 0.000019529*cos(Th5)*sin(Th4) - 0.0001116*sin(Th3)*sin(Th4) + 6.2e-9*sin(Th4)*sin(Th5) - 0.00002185*sin(Th4)*sin(Th6) + 0.00002185*cos(Th4)*cos(Th5)*cos(Th6) - 3.6e-6*cos(Th4)*cos(Th5)*sin(Th3) - 0.0033452*cos(Th4)*cos(Th5)*sin(Th5) - 0.0044118*cos(Th4)*sin(Th3)*sin(Th5) - 4.9934e-6*cos(Th5)*sin(Th4)*sin(Th6) - 0.0000207*sin(Th3)*sin(Th4)*sin(Th6) + 9.9869e-6*cos(Th4)*cos(Th5)^2*cos(Th6) + 0.0000207*cos(Th4)*cos(Th5)*cos(Th6)*sin(Th3) + 1.4868e-6*cos(Th6)*sin(Th4)*sin(Th5)*sin(Th6) - 1.4868e-6*cos(Th4)*cos(Th5)*cos(Th6)^2*sin(Th5))*dTh2*dTh4;
V425=(0.010487*sin(Th4) - 0.013381*cos(Th5)^2*sin(Th4) + 1.4868e-6*cos(Th6)^2*sin(Th4) - 1.86e-8*cos(Th4)*cos(Th5) - 0.000058586*cos(Th4)*sin(Th5) - 0.0046569*cos(Th5)*sin(Th4) + 3.8e-6*sin(Th4)*sin(Th5) - 5.9471e-6*cos(Th5)^2*cos(Th6)^2*sin(Th4) - 0.0044118*cos(Th5)*sin(Th3)*sin(Th4) - 1.216e-7*cos(Th5)*sin(Th4)*sin(Th5) - 0.00001498*cos(Th4)*sin(Th5)*sin(Th6) - 0.00002185*cos(Th6)*sin(Th4)*sin(Th5) + 3.6e-6*sin(Th3)*sin(Th4)*sin(Th5) - 4.4603e-6*cos(Th4)*cos(Th5)*cos(Th6)*sin(Th6) - 0.000039948*cos(Th5)*cos(Th6)*sin(Th4)*sin(Th5) - 0.0000207*cos(Th6)*sin(Th3)*sin(Th4)*sin(Th5))*dTh2*dTh5;
V426=(0.00002185*cos(Th4)*cos(Th6) - 0.00005504*cos(Th4)*sin(Th5) + 0.00001498*sin(Th4)*sin(Th6) - 0.000019974*cos(Th5)^2*sin(Th4)*sin(Th6) + 4.9934e-6*cos(Th4)*cos(Th5)*cos(Th6) + 0.0000207*cos(Th4)*cos(Th6)*sin(Th3) - 0.00002185*cos(Th5)*sin(Th4)*sin(Th6) - 5.9471e-6*cos(Th4)*cos(Th6)^2*sin(Th5) - 0.0000207*cos(Th5)*sin(Th3)*sin(Th4)*sin(Th6) + 5.9471e-6*cos(Th5)*cos(Th6)*sin(Th4)*sin(Th5)*sin(Th6))*dTh2*dTh6;
%---------------------------
V431=(0.5*(0.02603*cos(Th4)*sin(Th5) + 0.000115*sin(Th4)*sin(Th6) - 0.000115*cos(Th4)*cos(Th5)*cos(Th6))*(0.126*sin(Th2 + Th3) + 0.05206*sin(Th2 + Th3)*cos(Th5) + 0.254*cos(Th2)*sin(Th3) + 0.254*cos(Th3)*sin(Th2) + 0.05206*cos(Th2 + Th3)*cos(Th4)*sin(Th5) + 0.00023*cos(Th2 + Th3)*sin(Th4)*sin(Th6) + 0.00023*sin(Th2 + Th3)*cos(Th6)*sin(Th5) - 0.00023*cos(Th2 + Th3)*cos(Th4)*cos(Th5)*cos(Th6)) - 0.0051115*cos(Th2 + Th3) - 2.5e-11*cos(Th2 + Th3)*(23.0*cos(Th4)*sin(Th6) - 5206.0*sin(Th4)*sin(Th5) + 23.0*cos(Th5)*cos(Th6)*sin(Th4))^2 + 0.5*(0.00062*sin(Th4) + 0.00002*cos(Th4)*cos(Th5) - 0.00152*cos(Th4)*sin(Th5))*(0.126*sin(Th2 + Th3) + 0.00062*cos(Th2 + Th3)*sin(Th4) - 0.00152*sin(Th2 + Th3)*cos(Th5) - 0.00002*sin(Th2 + Th3)*sin(Th5) + 0.254*cos(Th2)*sin(Th3) + 0.254*cos(Th3)*sin(Th2) + 0.00002*cos(Th2 + Th3)*cos(Th4)*cos(Th5) - 0.00152*cos(Th2 + Th3)*cos(Th4)*sin(Th5)) + 0.010223*cos(Th2 + Th3)*cos(Th4)^2 + 0.0026665*cos(Th2 + Th3)*cos(Th5)^2 + 1.5e-6*cos(Th2 + Th3)*cos(Th6)^2 - 2.0e-10*cos(Th2 + Th3)*(31.0*cos(Th4) - 1.0*cos(Th5)*sin(Th4) + 76.0*sin(Th4)*sin(Th5))^2 + 2.0e-6*sin(Th2 + Th3)*cos(Th4)*cos(Th6) + 0.00002*sin(Th2 + Th3)*cos(Th5)*sin(Th4) - 0.005333*cos(Th2 + Th3)*cos(Th4)^2*cos(Th5)^2 - 3.0e-6*cos(Th2 + Th3)*cos(Th4)^2*cos(Th6)^2 + 1.5e-6*cos(Th2 + Th3)*cos(Th5)^2*cos(Th6)^2 + 4.0e-6*cos(Th2 + Th3)*cos(Th5)*cos(Th6)*sin(Th5) - 3.0e-6*cos(Th2 + Th3)*cos(Th4)^2*cos(Th5)^2*cos(Th6)^2 + 0.00008*cos(Th2 + Th3)*cos(Th4)*sin(Th4)*sin(Th5) + 0.0026665*sin(Th2 + Th3)*cos(Th4)*cos(Th5)*sin(Th5) + 2.0e-6*sin(Th2 + Th3)*cos(Th5)*sin(Th4)*sin(Th6) - 4.0e-6*sin(Th2 + Th3)*cos(Th4)*cos(Th5)^2*cos(Th6) - 8.0e-6*cos(Th2 + Th3)*cos(Th4)^2*cos(Th5)*cos(Th6)*sin(Th5) + 1.5e-6*sin(Th2 + Th3)*cos(Th4)*cos(Th5)*cos(Th6)^2*sin(Th5) + 8.0e-6*cos(Th2 + Th3)*cos(Th4)*sin(Th4)*sin(Th5)*sin(Th6) - 1.5e-6*sin(Th2 + Th3)*cos(Th6)*sin(Th4)*sin(Th5)*sin(Th6) + 6.0e-6*cos(Th2 + Th3)*cos(Th4)*cos(Th5)*cos(Th6)*sin(Th4)*sin(Th6))*dTh3*dTh1;
V432=(0.00579*sin(2.0*Th4) + 1.24e-8*cos(Th5) + 0.000039058*sin(Th5) - 2.48e-8*cos(Th4)^2*cos(Th5) - 0.000078115*cos(Th4)^2*sin(Th5) - 0.0001116*cos(Th3)*cos(Th4) + 9.9869e-6*sin(Th5)*sin(Th6) - 0.000019974*cos(Th4)^2*sin(Th5)*sin(Th6) + 3.6e-6*cos(Th3)*cos(Th5)*sin(Th4) - 0.0000207*cos(Th3)*cos(Th4)*sin(Th6) + 2.9736e-6*cos(Th5)*cos(Th6)*sin(Th6) + 0.0044118*cos(Th3)*sin(Th4)*sin(Th5) - 0.0066904*cos(Th4)*cos(Th5)^2*sin(Th4) - 2.9736e-6*cos(Th4)*cos(Th6)^2*sin(Th4) - 2.9736e-6*cos(Th4)*cos(Th5)^2*cos(Th6)^2*sin(Th4) - 0.0000207*cos(Th3)*cos(Th5)*cos(Th6)*sin(Th4) - 6.08e-8*cos(Th4)*cos(Th5)*sin(Th4)*sin(Th5) - 5.9471e-6*cos(Th4)^2*cos(Th5)*cos(Th6)*sin(Th6) - 0.000019974*cos(Th4)*cos(Th5)*cos(Th6)*sin(Th4)*sin(Th5))*dTh3*dTh2;
V433=(0.00579*sin(2.0*Th4) + 1.24e-8*cos(Th5) + 0.000039058*sin(Th5) - 2.48e-8*cos(Th4)^2*cos(Th5) - 0.000078115*cos(Th4)^2*sin(Th5) + 9.9869e-6*sin(Th5)*sin(Th6) - 0.000019974*cos(Th4)^2*sin(Th5)*sin(Th6) + 2.9736e-6*cos(Th5)*cos(Th6)*sin(Th6) - 0.0066904*cos(Th4)*cos(Th5)^2*sin(Th4) - 2.9736e-6*cos(Th4)*cos(Th6)^2*sin(Th4) - 2.9736e-6*cos(Th4)*cos(Th5)^2*cos(Th6)^2*sin(Th4) - 6.08e-8*cos(Th4)*cos(Th5)*sin(Th4)*sin(Th5) - 5.9471e-6*cos(Th4)^2*cos(Th5)*cos(Th6)*sin(Th6) - 0.000019974*cos(Th4)*cos(Th5)*cos(Th6)*sin(Th4)*sin(Th5))*dTh3*dTh3;
V434=(3.04e-8*cos(Th4)*cos(Th5)^2 - 0.0001178*sin(Th4) - 1.52e-8*cos(Th4) - 3.8e-6*cos(Th4)*cos(Th5) - 4.9934e-6*cos(Th4)*cos(Th6) - 0.0046569*cos(Th4)*sin(Th5) - 0.000019529*cos(Th5)*sin(Th4) + 6.2e-9*sin(Th4)*sin(Th5) - 0.00002185*sin(Th4)*sin(Th6) + 0.00002185*cos(Th4)*cos(Th5)*cos(Th6) - 0.0033452*cos(Th4)*cos(Th5)*sin(Th5) - 4.9934e-6*cos(Th5)*sin(Th4)*sin(Th6) + 9.9869e-6*cos(Th4)*cos(Th5)^2*cos(Th6) + 1.4868e-6*cos(Th6)*sin(Th4)*sin(Th5)*sin(Th6) - 1.4868e-6*cos(Th4)*cos(Th5)*cos(Th6)^2*sin(Th5))*dTh3*dTh4;
V435=(0.010487*sin(Th4) - 0.013381*cos(Th5)^2*sin(Th4) + 1.4868e-6*cos(Th6)^2*sin(Th4) - 1.86e-8*cos(Th4)*cos(Th5) - 0.000058586*cos(Th4)*sin(Th5) - 0.0046569*cos(Th5)*sin(Th4) + 3.8e-6*sin(Th4)*sin(Th5) - 5.9471e-6*cos(Th5)^2*cos(Th6)^2*sin(Th4) - 1.216e-7*cos(Th5)*sin(Th4)*sin(Th5) - 0.00001498*cos(Th4)*sin(Th5)*sin(Th6) - 0.00002185*cos(Th6)*sin(Th4)*sin(Th5) - 4.4603e-6*cos(Th4)*cos(Th5)*cos(Th6)*sin(Th6) - 0.000039948*cos(Th5)*cos(Th6)*sin(Th4)*sin(Th5))*dTh3*dTh5;
V436=(0.00002185*cos(Th4)*cos(Th6) - 0.00005504*cos(Th4)*sin(Th5) + 0.00001498*sin(Th4)*sin(Th6) - 0.000019974*cos(Th5)^2*sin(Th4)*sin(Th6) + 4.9934e-6*cos(Th4)*cos(Th5)*cos(Th6) - 0.00002185*cos(Th5)*sin(Th4)*sin(Th6) - 5.9471e-6*cos(Th4)*cos(Th6)^2*sin(Th5) + 5.9471e-6*cos(Th5)*cos(Th6)*sin(Th4)*sin(Th5)*sin(Th6))*dTh3*dTh6;
%---------------------------
V441=(0.0000217*cos(Th4) - 0.0001116*cos(Th4)*sin(Th2) - 7.0e-7*cos(Th5)*sin(Th4) + 4.025e-6*cos(Th4)*sin(Th6) - 0.00085785*sin(Th4)*sin(Th5) + 0.0001178*cos(Th2)*cos(Th3)*cos(Th4) - 1.52e-8*cos(Th2)*cos(Th3)*sin(Th4) + 4.025e-6*cos(Th5)*cos(Th6)*sin(Th4) - 0.0001178*cos(Th4)*sin(Th2)*sin(Th3) + 3.6e-6*cos(Th5)*sin(Th2)*sin(Th4) - 0.0000207*cos(Th4)*sin(Th2)*sin(Th6) + 1.52e-8*sin(Th2)*sin(Th3)*sin(Th4) + 0.0044118*sin(Th2)*sin(Th4)*sin(Th5) + 0.000019529*cos(Th2)*cos(Th3)*cos(Th4)*cos(Th5) - 6.2e-9*cos(Th2)*cos(Th3)*cos(Th4)*sin(Th5) - 3.8e-6*cos(Th2)*cos(Th3)*cos(Th5)*sin(Th4) + 0.00002185*cos(Th2)*cos(Th3)*cos(Th4)*sin(Th6) - 4.9934e-6*cos(Th2)*cos(Th3)*cos(Th6)*sin(Th4) - 0.0046569*cos(Th2)*cos(Th3)*sin(Th4)*sin(Th5) - 0.000019529*cos(Th4)*cos(Th5)*sin(Th2)*sin(Th3) - 0.0000207*cos(Th5)*cos(Th6)*sin(Th2)*sin(Th4) + 6.2e-9*cos(Th4)*sin(Th2)*sin(Th3)*sin(Th5) + 3.8e-6*cos(Th5)*sin(Th2)*sin(Th3)*sin(Th4) - 0.00002185*cos(Th4)*sin(Th2)*sin(Th3)*sin(Th6) + 4.9934e-6*cos(Th6)*sin(Th2)*sin(Th3)*sin(Th4) + 0.0046569*sin(Th2)*sin(Th3)*sin(Th4)*sin(Th5) + 3.04e-8*cos(Th2)*cos(Th3)*cos(Th5)^2*sin(Th4) - 3.04e-8*cos(Th5)^2*sin(Th2)*sin(Th3)*sin(Th4) + 4.9934e-6*cos(Th2)*cos(Th3)*cos(Th4)*cos(Th5)*sin(Th6) + 0.00002185*cos(Th2)*cos(Th3)*cos(Th5)*cos(Th6)*sin(Th4) - 0.0033452*cos(Th2)*cos(Th3)*cos(Th5)*sin(Th4)*sin(Th5) - 4.9934e-6*cos(Th4)*cos(Th5)*sin(Th2)*sin(Th3)*sin(Th6) - 0.00002185*cos(Th5)*cos(Th6)*sin(Th2)*sin(Th3)*sin(Th4) + 0.0033452*cos(Th5)*sin(Th2)*sin(Th3)*sin(Th4)*sin(Th5) + 9.9869e-6*cos(Th2)*cos(Th3)*cos(Th5)^2*cos(Th6)*sin(Th4) - 9.9869e-6*cos(Th5)^2*cos(Th6)*sin(Th2)*sin(Th3)*sin(Th4) - 1.4868e-6*cos(Th2)*cos(Th3)*cos(Th5)*cos(Th6)^2*sin(Th4)*sin(Th5) + 1.4868e-6*cos(Th5)*cos(Th6)^2*sin(Th2)*sin(Th3)*sin(Th4)*sin(Th5) - 1.4868e-6*cos(Th2)*cos(Th3)*cos(Th4)*cos(Th6)*sin(Th5)*sin(Th6) + 1.4868e-6*cos(Th4)*cos(Th6)*sin(Th2)*sin(Th3)*sin(Th5)*sin(Th6))*dTh4*dTh1;
V442=(1.52e-8*cos(Th4) + 0.0001178*sin(Th4) - 3.04e-8*cos(Th4)*cos(Th5)^2 + 3.8e-6*cos(Th4)*cos(Th5) + 4.9934e-6*cos(Th4)*cos(Th6) + 0.0046569*cos(Th4)*sin(Th5) + 0.000019529*cos(Th5)*sin(Th4) + 0.0001116*sin(Th3)*sin(Th4) - 6.2e-9*sin(Th4)*sin(Th5) + 0.00002185*sin(Th4)*sin(Th6) - 0.00002185*cos(Th4)*cos(Th5)*cos(Th6) + 3.6e-6*cos(Th4)*cos(Th5)*sin(Th3) + 0.0033452*cos(Th4)*cos(Th5)*sin(Th5) + 0.0044118*cos(Th4)*sin(Th3)*sin(Th5) + 4.9934e-6*cos(Th5)*sin(Th4)*sin(Th6) + 0.0000207*sin(Th3)*sin(Th4)*sin(Th6) - 9.9869e-6*cos(Th4)*cos(Th5)^2*cos(Th6) - 0.0000207*cos(Th4)*cos(Th5)*cos(Th6)*sin(Th3) - 1.4868e-6*cos(Th6)*sin(Th4)*sin(Th5)*sin(Th6) + 1.4868e-6*cos(Th4)*cos(Th5)*cos(Th6)^2*sin(Th5))*dTh4*dTh2;
V443=(1.52e-8*cos(Th4) + 0.0001178*sin(Th4) - 3.04e-8*cos(Th4)*cos(Th5)^2 + 3.8e-6*cos(Th4)*cos(Th5) + 4.9934e-6*cos(Th4)*cos(Th6) + 0.0046569*cos(Th4)*sin(Th5) + 0.000019529*cos(Th5)*sin(Th4) - 6.2e-9*sin(Th4)*sin(Th5) + 0.00002185*sin(Th4)*sin(Th6) - 8.0e-10*cos(Th2 + Th3)*sin(Th2 + Th3)*(31.0*cos(Th4) - 1.0*cos(Th5)*sin(Th4) + 76.0*sin(Th4)*sin(Th5))^2 - 0.00002185*cos(Th4)*cos(Th5)*cos(Th6) + 0.0033452*cos(Th4)*cos(Th5)*sin(Th5) + 4.9934e-6*cos(Th5)*sin(Th4)*sin(Th6) - 1.0e-10*cos(Th2 + Th3)*sin(Th2 + Th3)*(23.0*cos(Th4)*sin(Th6) - 5206.0*sin(Th4)*sin(Th5) + 23.0*cos(Th5)*cos(Th6)*sin(Th4))^2 - 9.9869e-6*cos(Th4)*cos(Th5)^2*cos(Th6) - 2.0*cos(Th2 + Th3)*cos(Th1)*(0.00062*cos(Th4) - 0.00002*cos(Th5)*sin(Th4) + 0.00152*sin(Th4)*sin(Th5))*(0.00062*sin(Th1)*sin(Th4) - 0.00062*sin(Th2 + Th3)*cos(Th1)*cos(Th4) + 0.00002*cos(Th4)*cos(Th5)*sin(Th1) - 0.00152*cos(Th4)*sin(Th1)*sin(Th5) + 0.00002*sin(Th2 + Th3)*cos(Th1)*cos(Th5)*sin(Th4) - 0.00152*sin(Th2 + Th3)*cos(Th1)*sin(Th4)*sin(Th5)) - 1.4868e-6*cos(Th6)*sin(Th4)*sin(Th5)*sin(Th6) + 1.4868e-6*cos(Th4)*cos(Th5)*cos(Th6)^2*sin(Th5) - 1.0*cos(Th2 + Th3)*cos(Th1)*(0.00023*cos(Th4)*sin(Th6) - 0.05206*sin(Th4)*sin(Th5) + 0.00023*cos(Th5)*cos(Th6)*sin(Th4))*(0.05206*cos(Th4)*sin(Th1)*sin(Th5) + 0.00023*sin(Th1)*sin(Th4)*sin(Th6) - 0.00023*sin(Th2 + Th3)*cos(Th1)*cos(Th4)*sin(Th6) + 0.05206*sin(Th2 + Th3)*cos(Th1)*sin(Th4)*sin(Th5) - 0.00023*cos(Th4)*cos(Th5)*cos(Th6)*sin(Th1) - 0.00023*sin(Th2 + Th3)*cos(Th1)*cos(Th5)*cos(Th6)*sin(Th4)) + cos(Th2 + Th3)*sin(Th1)*(0.00023*cos(Th4)*sin(Th6) - 0.05206*sin(Th4)*sin(Th5) + 0.00023*cos(Th5)*cos(Th6)*sin(Th4))*(0.05206*cos(Th1)*cos(Th4)*sin(Th5) + 0.00023*cos(Th1)*sin(Th4)*sin(Th6) + 0.00023*sin(Th2 + Th3)*cos(Th4)*sin(Th1)*sin(Th6) - 0.05206*sin(Th2 + Th3)*sin(Th1)*sin(Th4)*sin(Th5) - 0.00023*cos(Th1)*cos(Th4)*cos(Th5)*cos(Th6) + 0.00023*sin(Th2 + Th3)*cos(Th5)*cos(Th6)*sin(Th1)*sin(Th4)) + 2.0*cos(Th2 + Th3)*sin(Th1)*(0.00062*cos(Th4) - 0.00002*cos(Th5)*sin(Th4) + 0.00152*sin(Th4)*sin(Th5))*(0.00062*cos(Th1)*sin(Th4) + 0.00062*sin(Th2 + Th3)*cos(Th4)*sin(Th1) + 0.00002*cos(Th1)*cos(Th4)*cos(Th5) - 0.00152*cos(Th1)*cos(Th4)*sin(Th5) - 0.00002*sin(Th2 + Th3)*cos(Th5)*sin(Th1)*sin(Th4) + 0.00152*sin(Th2 + Th3)*sin(Th1)*sin(Th4)*sin(Th5)))*dTh4*dTh3;
V444=(0)*dTh4*dTh4;
V445=(0.000019974*cos(Th6) - 1.216e-7*cos(Th5)^2 - 0.000039948*cos(Th5)^2*cos(Th6) + 0.013381*cos(Th5)*sin(Th5) + 5.9471e-6*cos(Th5)*cos(Th6)^2*sin(Th5) + 6.08e-8)*dTh4*dTh5;
V446=(1.6941e-26*sin(Th6)*(5.8952e20*sin(2.0*Th5) - 3.5105e20*cos(Th6) + 3.5105e20*cos(Th5)^2*cos(Th6)))*dTh4*dTh6;
%---------------------------
V451=(0.00085785*cos(Th4)*cos(Th5) - 7.0e-7*cos(Th4)*sin(Th5) + 0.0037962*cos(Th2)*cos(Th3)*cos(Th4) - 0.0044118*cos(Th4)*cos(Th5)*sin(Th2) + 4.025e-6*cos(Th4)*cos(Th6)*sin(Th5) - 0.0037962*cos(Th4)*sin(Th2)*sin(Th3) + 3.6e-6*cos(Th4)*sin(Th2)*sin(Th5) + 0.0046569*cos(Th2)*cos(Th3)*cos(Th4)*cos(Th5) - 3.8e-6*cos(Th2)*cos(Th3)*cos(Th4)*sin(Th5) + 6.2e-9*cos(Th2)*cos(Th3)*cos(Th5)*sin(Th4) + 0.000019529*cos(Th2)*cos(Th3)*sin(Th4)*sin(Th5) - 0.0046569*cos(Th4)*cos(Th5)*sin(Th2)*sin(Th3) - 0.0000207*cos(Th4)*cos(Th6)*sin(Th2)*sin(Th5) + 3.8e-6*cos(Th4)*sin(Th2)*sin(Th3)*sin(Th5) - 6.2e-9*cos(Th5)*sin(Th2)*sin(Th3)*sin(Th4) - 0.000019529*sin(Th2)*sin(Th3)*sin(Th4)*sin(Th5) - 1.4868e-6*cos(Th2)*cos(Th3)*cos(Th4)*cos(Th6)^2 + 1.4868e-6*cos(Th4)*cos(Th6)^2*sin(Th2)*sin(Th3) + 0.00002185*cos(Th2)*cos(Th3)*cos(Th4)*cos(Th6)*sin(Th5) + 4.9934e-6*cos(Th2)*cos(Th3)*sin(Th4)*sin(Th5)*sin(Th6) - 0.00002185*cos(Th4)*cos(Th6)*sin(Th2)*sin(Th3)*sin(Th5) - 4.9934e-6*sin(Th2)*sin(Th3)*sin(Th4)*sin(Th5)*sin(Th6) + 1.4868e-6*cos(Th2)*cos(Th3)*cos(Th5)*cos(Th6)*sin(Th4)*sin(Th6) - 1.4868e-6*cos(Th5)*cos(Th6)*sin(Th2)*sin(Th3)*sin(Th4)*sin(Th6))*dTh5*dTh1;
V452=(0.0037962*sin(Th4) - 1.4868e-6*cos(Th6)^2*sin(Th4) - 6.2e-9*cos(Th4)*cos(Th5) - 0.000019529*cos(Th4)*sin(Th5) + 0.0046569*cos(Th5)*sin(Th4) - 3.8e-6*sin(Th4)*sin(Th5) + 0.0044118*cos(Th5)*sin(Th3)*sin(Th4) - 4.9934e-6*cos(Th4)*sin(Th5)*sin(Th6) + 0.00002185*cos(Th6)*sin(Th4)*sin(Th5) - 3.6e-6*sin(Th3)*sin(Th4)*sin(Th5) - 1.4868e-6*cos(Th4)*cos(Th5)*cos(Th6)*sin(Th6) + 0.0000207*cos(Th6)*sin(Th3)*sin(Th4)*sin(Th5))*dTh5*dTh2;
V453=(0.0037962*sin(Th4) - 1.4868e-6*cos(Th6)^2*sin(Th4) - 6.2e-9*cos(Th4)*cos(Th5) - 0.000019529*cos(Th4)*sin(Th5) + 0.0046569*cos(Th5)*sin(Th4) - 3.8e-6*sin(Th4)*sin(Th5) + sin(Th2 + Th3)*(0.00062*cos(Th4) - 0.00002*cos(Th5)*sin(Th4) + 0.00152*sin(Th4)*sin(Th5))*(0.00002*sin(Th2 + Th3)*cos(Th5) - 0.00152*sin(Th2 + Th3)*sin(Th5) + 0.00152*cos(Th2 + Th3)*cos(Th4)*cos(Th5) + 0.00002*cos(Th2 + Th3)*cos(Th4)*sin(Th5)) + cos(Th2 + Th3)*(0.00062*cos(Th4) - 0.00002*cos(Th5)*sin(Th4) + 0.00152*sin(Th4)*sin(Th5))*(0.00152*cos(Th2 + Th3)*sin(Th5) - 0.00002*cos(Th2 + Th3)*cos(Th5) + 0.00152*sin(Th2 + Th3)*cos(Th4)*cos(Th5) + 0.00002*sin(Th2 + Th3)*cos(Th4)*sin(Th5)) - 0.5*cos(Th2 + Th3)*(0.00023*cos(Th4)*sin(Th6) - 0.05206*sin(Th4)*sin(Th5) + 0.00023*cos(Th5)*cos(Th6)*sin(Th4))*(0.05206*cos(Th2 + Th3)*sin(Th5) - 0.00023*cos(Th2 + Th3)*cos(Th5)*cos(Th6) + 0.05206*sin(Th2 + Th3)*cos(Th4)*cos(Th5) + 0.00023*sin(Th2 + Th3)*cos(Th4)*cos(Th6)*sin(Th5)) - 0.5*cos(Th1)*(0.05206*cos(Th2 + Th3)*cos(Th4)*cos(Th5) - 0.05206*sin(Th2 + Th3)*sin(Th5) + 0.00023*sin(Th2 + Th3)*cos(Th5)*cos(Th6) + 0.00023*cos(Th2 + Th3)*cos(Th4)*cos(Th6)*sin(Th5))*(0.05206*cos(Th4)*sin(Th1)*sin(Th5) + 0.00023*sin(Th1)*sin(Th4)*sin(Th6) - 0.00023*sin(Th2 + Th3)*cos(Th1)*cos(Th4)*sin(Th6) + 0.05206*sin(Th2 + Th3)*cos(Th1)*sin(Th4)*sin(Th5) - 0.00023*cos(Th4)*cos(Th5)*cos(Th6)*sin(Th1) - 0.00023*sin(Th2 + Th3)*cos(Th1)*cos(Th5)*cos(Th6)*sin(Th4)) - 1.0*sin(Th1)*(0.00002*sin(Th2 + Th3)*cos(Th5) - 0.00152*sin(Th2 + Th3)*sin(Th5) + 0.00152*cos(Th2 + Th3)*cos(Th4)*cos(Th5) + 0.00002*cos(Th2 + Th3)*cos(Th4)*sin(Th5))*(0.00062*cos(Th1)*sin(Th4) + 0.00062*sin(Th2 + Th3)*cos(Th4)*sin(Th1) + 0.00002*cos(Th1)*cos(Th4)*cos(Th5) - 0.00152*cos(Th1)*cos(Th4)*sin(Th5) - 0.00002*sin(Th2 + Th3)*cos(Th5)*sin(Th1)*sin(Th4) + 0.00152*sin(Th2 + Th3)*sin(Th1)*sin(Th4)*sin(Th5)) + 0.5*sin(Th1)*(0.05206*cos(Th2 + Th3)*cos(Th4)*cos(Th5) - 0.05206*sin(Th2 + Th3)*sin(Th5) + 0.00023*sin(Th2 + Th3)*cos(Th5)*cos(Th6) + 0.00023*cos(Th2 + Th3)*cos(Th4)*cos(Th6)*sin(Th5))*(0.05206*cos(Th1)*cos(Th4)*sin(Th5) + 0.00023*cos(Th1)*sin(Th4)*sin(Th6) + 0.00023*sin(Th2 + Th3)*cos(Th4)*sin(Th1)*sin(Th6) - 0.05206*sin(Th2 + Th3)*sin(Th1)*sin(Th4)*sin(Th5) - 0.00023*cos(Th1)*cos(Th4)*cos(Th5)*cos(Th6) + 0.00023*sin(Th2 + Th3)*cos(Th5)*cos(Th6)*sin(Th1)*sin(Th4)) - 0.5*sin(Th2 + Th3)*(0.00023*cos(Th4)*sin(Th6) - 0.05206*sin(Th4)*sin(Th5) + 0.00023*cos(Th5)*cos(Th6)*sin(Th4))*(0.05206*cos(Th2 + Th3)*cos(Th4)*cos(Th5) - 0.05206*sin(Th2 + Th3)*sin(Th5) + 0.00023*sin(Th2 + Th3)*cos(Th5)*cos(Th6) + 0.00023*cos(Th2 + Th3)*cos(Th4)*cos(Th6)*sin(Th5)) - 4.9934e-6*cos(Th4)*sin(Th5)*sin(Th6) + 0.00002185*cos(Th6)*sin(Th4)*sin(Th5) + cos(Th1)*(0.00002*sin(Th2 + Th3)*cos(Th5) - 0.00152*sin(Th2 + Th3)*sin(Th5) + 0.00152*cos(Th2 + Th3)*cos(Th4)*cos(Th5) + 0.00002*cos(Th2 + Th3)*cos(Th4)*sin(Th5))*(0.00062*sin(Th1)*sin(Th4) - 0.00062*sin(Th2 + Th3)*cos(Th1)*cos(Th4) + 0.00002*cos(Th4)*cos(Th5)*sin(Th1) - 0.00152*cos(Th4)*sin(Th1)*sin(Th5) + 0.00002*sin(Th2 + Th3)*cos(Th1)*cos(Th5)*sin(Th4) - 0.00152*sin(Th2 + Th3)*cos(Th1)*sin(Th4)*sin(Th5)) - 1.0*cos(Th2 + Th3)*sin(Th1)*(0.00062*cos(Th4) - 0.00002*cos(Th5)*sin(Th4) + 0.00152*sin(Th4)*sin(Th5))*(0.00152*cos(Th2 + Th3)*sin(Th1)*sin(Th5) - 0.00002*cos(Th2 + Th3)*cos(Th5)*sin(Th1) + 0.00152*cos(Th1)*cos(Th5)*sin(Th4) + 0.00002*cos(Th1)*sin(Th4)*sin(Th5) + 0.00152*sin(Th2 + Th3)*cos(Th4)*cos(Th5)*sin(Th1) + 0.00002*sin(Th2 + Th3)*cos(Th4)*sin(Th1)*sin(Th5)) + 0.5*cos(Th2 + Th3)*sin(Th1)*(0.00023*cos(Th4)*sin(Th6) - 0.05206*sin(Th4)*sin(Th5) + 0.00023*cos(Th5)*cos(Th6)*sin(Th4))*(0.05206*cos(Th2 + Th3)*sin(Th1)*sin(Th5) + 0.05206*cos(Th1)*cos(Th5)*sin(Th4) - 0.00023*cos(Th2 + Th3)*cos(Th5)*cos(Th6)*sin(Th1) + 0.05206*sin(Th2 + Th3)*cos(Th4)*cos(Th5)*sin(Th1) + 0.00023*cos(Th1)*cos(Th6)*sin(Th4)*sin(Th5) + 0.00023*sin(Th2 + Th3)*cos(Th4)*cos(Th6)*sin(Th1)*sin(Th5)) + 0.5*cos(Th2 + Th3)*cos(Th1)*(0.00023*cos(Th4)*sin(Th6) - 0.05206*sin(Th4)*sin(Th5) + 0.00023*cos(Th5)*cos(Th6)*sin(Th4))*(0.05206*cos(Th2 + Th3)*cos(Th1)*sin(Th5) - 0.05206*cos(Th5)*sin(Th1)*sin(Th4) + 0.05206*sin(Th2 + Th3)*cos(Th1)*cos(Th4)*cos(Th5) - 0.00023*cos(Th6)*sin(Th1)*sin(Th4)*sin(Th5) - 0.00023*cos(Th2 + Th3)*cos(Th1)*cos(Th5)*cos(Th6) + 0.00023*sin(Th2 + Th3)*cos(Th1)*cos(Th4)*cos(Th6)*sin(Th5)) - 1.4868e-6*cos(Th4)*cos(Th5)*cos(Th6)*sin(Th6) + cos(Th2 + Th3)*cos(Th1)*(0.00062*cos(Th4) - 0.00002*cos(Th5)*sin(Th4) + 0.00152*sin(Th4)*sin(Th5))*(0.00002*cos(Th2 + Th3)*cos(Th1)*cos(Th5) - 0.00152*cos(Th2 + Th3)*cos(Th1)*sin(Th5) + 0.00152*cos(Th5)*sin(Th1)*sin(Th4) + 0.00002*sin(Th1)*sin(Th4)*sin(Th5) - 0.00152*sin(Th2 + Th3)*cos(Th1)*cos(Th4)*cos(Th5) - 0.00002*sin(Th2 + Th3)*cos(Th1)*cos(Th4)*sin(Th5)))*dTh5*dTh3;
V454=(0.5*(0.00023*cos(Th1)*cos(Th4)*sin(Th6) - 0.05206*cos(Th1)*sin(Th4)*sin(Th5) - 0.05206*sin(Th2 + Th3)*cos(Th4)*sin(Th1)*sin(Th5) - 0.00023*sin(Th2 + Th3)*sin(Th1)*sin(Th4)*sin(Th6) + 0.00023*cos(Th1)*cos(Th5)*cos(Th6)*sin(Th4) + 0.00023*sin(Th2 + Th3)*cos(Th4)*cos(Th5)*cos(Th6)*sin(Th1))*(0.02603*cos(Th2 + Th3)*sin(Th1)*sin(Th5) + 0.02603*cos(Th1)*cos(Th5)*sin(Th4) - 0.000115*cos(Th2 + Th3)*cos(Th5)*cos(Th6)*sin(Th1) + 0.02603*sin(Th2 + Th3)*cos(Th4)*cos(Th5)*sin(Th1) + 0.000115*cos(Th1)*cos(Th6)*sin(Th4)*sin(Th5) + 0.000115*sin(Th2 + Th3)*cos(Th4)*cos(Th6)*sin(Th1)*sin(Th5)) - 0.5*(0.00062*cos(Th1)*cos(Th4) - 0.00062*sin(Th2 + Th3)*sin(Th1)*sin(Th4) - 0.00002*cos(Th1)*cos(Th5)*sin(Th4) + 0.00152*cos(Th1)*sin(Th4)*sin(Th5) - 0.00002*sin(Th2 + Th3)*cos(Th4)*cos(Th5)*sin(Th1) + 0.00152*sin(Th2 + Th3)*cos(Th4)*sin(Th1)*sin(Th5))*(0.00152*cos(Th2 + Th3)*sin(Th1)*sin(Th5) - 0.00002*cos(Th2 + Th3)*cos(Th5)*sin(Th1) + 0.00152*cos(Th1)*cos(Th5)*sin(Th4) + 0.00002*cos(Th1)*sin(Th4)*sin(Th5) + 0.00152*sin(Th2 + Th3)*cos(Th4)*cos(Th5)*sin(Th1) + 0.00002*sin(Th2 + Th3)*cos(Th4)*sin(Th1)*sin(Th5)) - 0.5*(0.05206*cos(Th2 + Th3)*cos(Th1)*sin(Th5) - 0.05206*cos(Th5)*sin(Th1)*sin(Th4) + 0.05206*sin(Th2 + Th3)*cos(Th1)*cos(Th4)*cos(Th5) - 0.00023*cos(Th6)*sin(Th1)*sin(Th4)*sin(Th5) - 0.00023*cos(Th2 + Th3)*cos(Th1)*cos(Th5)*cos(Th6) + 0.00023*sin(Th2 + Th3)*cos(Th1)*cos(Th4)*cos(Th6)*sin(Th5))*(0.000115*cos(Th4)*sin(Th1)*sin(Th6) - 0.02603*sin(Th1)*sin(Th4)*sin(Th5) + 0.02603*sin(Th2 + Th3)*cos(Th1)*cos(Th4)*sin(Th5) + 0.000115*sin(Th2 + Th3)*cos(Th1)*sin(Th4)*sin(Th6) + 0.000115*cos(Th5)*cos(Th6)*sin(Th1)*sin(Th4) - 0.000115*sin(Th2 + Th3)*cos(Th1)*cos(Th4)*cos(Th5)*cos(Th6)) - 0.5*(0.00002*cos(Th2 + Th3)*cos(Th1)*cos(Th5) - 0.00152*cos(Th2 + Th3)*cos(Th1)*sin(Th5) + 0.00152*cos(Th5)*sin(Th1)*sin(Th4) + 0.00002*sin(Th1)*sin(Th4)*sin(Th5) - 0.00152*sin(Th2 + Th3)*cos(Th1)*cos(Th4)*cos(Th5) - 0.00002*sin(Th2 + Th3)*cos(Th1)*cos(Th4)*sin(Th5))*(0.00062*cos(Th4)*sin(Th1) + 0.00062*sin(Th2 + Th3)*cos(Th1)*sin(Th4) - 0.00002*cos(Th5)*sin(Th1)*sin(Th4) + 0.00152*sin(Th1)*sin(Th4)*sin(Th5) + 0.00002*sin(Th2 + Th3)*cos(Th1)*cos(Th4)*cos(Th5) - 0.00152*sin(Th2 + Th3)*cos(Th1)*cos(Th4)*sin(Th5)) + 0.5*cos(Th2 + Th3)*(0.00062*sin(Th4) + 0.00002*cos(Th4)*cos(Th5) - 0.00152*cos(Th4)*sin(Th5))*(0.00002*sin(Th2 + Th3)*cos(Th5) - 0.00152*sin(Th2 + Th3)*sin(Th5) + 0.00152*cos(Th2 + Th3)*cos(Th4)*cos(Th5) + 0.00002*cos(Th2 + Th3)*cos(Th4)*sin(Th5)) + 0.5*(0.05206*cos(Th5) + 0.00023*cos(Th6)*sin(Th5))*(0.5*cos(Th1)*cos(Th4) - 0.5*sin(Th2 + Th3)*sin(Th1)*sin(Th4))*(0.05206*cos(Th1)*cos(Th4)*sin(Th5) + 0.00023*cos(Th1)*sin(Th4)*sin(Th6) + 0.00023*sin(Th2 + Th3)*cos(Th4)*sin(Th1)*sin(Th6) - 0.05206*sin(Th2 + Th3)*sin(Th1)*sin(Th4)*sin(Th5) - 0.00023*cos(Th1)*cos(Th4)*cos(Th5)*cos(Th6) + 0.00023*sin(Th2 + Th3)*cos(Th5)*cos(Th6)*sin(Th1)*sin(Th4)) - 0.5*(0.00152*cos(Th5) + 0.00002*sin(Th5))*(cos(Th4)*sin(Th1) + sin(Th2 + Th3)*cos(Th1)*sin(Th4))*(0.00062*sin(Th1)*sin(Th4) - 0.00062*sin(Th2 + Th3)*cos(Th1)*cos(Th4) + 0.00002*cos(Th4)*cos(Th5)*sin(Th1) - 0.00152*cos(Th4)*sin(Th1)*sin(Th5) + 0.00002*sin(Th2 + Th3)*cos(Th1)*cos(Th5)*sin(Th4) - 0.00152*sin(Th2 + Th3)*cos(Th1)*sin(Th4)*sin(Th5)) - 0.25*cos(Th2 + Th3)*(0.05206*cos(Th4)*sin(Th5) + 0.00023*sin(Th4)*sin(Th6) - 0.00023*cos(Th4)*cos(Th5)*cos(Th6))*(0.05206*cos(Th2 + Th3)*cos(Th4)*cos(Th5) - 0.05206*sin(Th2 + Th3)*sin(Th5) + 0.00023*sin(Th2 + Th3)*cos(Th5)*cos(Th6) + 0.00023*cos(Th2 + Th3)*cos(Th4)*cos(Th6)*sin(Th5)) + 0.5*(0.5*cos(Th4)*sin(Th1) + 0.5*sin(Th2 + Th3)*cos(Th1)*sin(Th4))*(0.05206*cos(Th5) + 0.00023*cos(Th6)*sin(Th5))*(0.05206*cos(Th4)*sin(Th1)*sin(Th5) + 0.00023*sin(Th1)*sin(Th4)*sin(Th6) - 0.00023*sin(Th2 + Th3)*cos(Th1)*cos(Th4)*sin(Th6) + 0.05206*sin(Th2 + Th3)*cos(Th1)*sin(Th4)*sin(Th5) - 0.00023*cos(Th4)*cos(Th5)*cos(Th6)*sin(Th1) - 0.00023*sin(Th2 + Th3)*cos(Th1)*cos(Th5)*cos(Th6)*sin(Th4)) - 0.5*(0.00152*cos(Th5) + 0.00002*sin(Th5))*(cos(Th1)*cos(Th4) - 1.0*sin(Th2 + Th3)*sin(Th1)*sin(Th4))*(0.00062*cos(Th1)*sin(Th4) + 0.00062*sin(Th2 + Th3)*cos(Th4)*sin(Th1) + 0.00002*cos(Th1)*cos(Th4)*cos(Th5) - 0.00152*cos(Th1)*cos(Th4)*sin(Th5) - 0.00002*sin(Th2 + Th3)*cos(Th5)*sin(Th1)*sin(Th4) + 0.00152*sin(Th2 + Th3)*sin(Th1)*sin(Th4)*sin(Th5)) - 0.25*cos(Th2 + Th3)^2*sin(Th4)*(0.05206*cos(Th5) + 0.00023*cos(Th6)*sin(Th5))*(0.00023*cos(Th4)*sin(Th6) - 0.05206*sin(Th4)*sin(Th5) + 0.00023*cos(Th5)*cos(Th6)*sin(Th4)) + 0.5*cos(Th2 + Th3)^2*sin(Th4)*(0.00152*cos(Th5) + 0.00002*sin(Th5))*(0.00062*cos(Th4) - 0.00002*cos(Th5)*sin(Th4) + 0.00152*sin(Th4)*sin(Th5)))*dTh5*dTh4;
V455=((0.00152*cos(Th2 + Th3)*cos(Th1)*cos(Th5) + 0.00002*cos(Th2 + Th3)*cos(Th1)*sin(Th5) - 0.00002*cos(Th5)*sin(Th1)*sin(Th4) + 0.00152*sin(Th1)*sin(Th4)*sin(Th5) + 0.00002*sin(Th2 + Th3)*cos(Th1)*cos(Th4)*cos(Th5) - 0.00152*sin(Th2 + Th3)*cos(Th1)*cos(Th4)*sin(Th5))*(0.00062*sin(Th1)*sin(Th4) - 0.00062*sin(Th2 + Th3)*cos(Th1)*cos(Th4) + 0.00002*cos(Th4)*cos(Th5)*sin(Th1) - 0.00152*cos(Th4)*sin(Th1)*sin(Th5) + 0.00002*sin(Th2 + Th3)*cos(Th1)*cos(Th5)*sin(Th4) - 0.00152*sin(Th2 + Th3)*cos(Th1)*sin(Th4)*sin(Th5)) - 1.0*(0.00152*cos(Th2 + Th3)*cos(Th5)*sin(Th1) + 0.00002*cos(Th2 + Th3)*sin(Th1)*sin(Th5) + 0.00002*cos(Th1)*cos(Th5)*sin(Th4) - 0.00152*cos(Th1)*sin(Th4)*sin(Th5) + 0.00002*sin(Th2 + Th3)*cos(Th4)*cos(Th5)*sin(Th1) - 0.00152*sin(Th2 + Th3)*cos(Th4)*sin(Th1)*sin(Th5))*(0.00062*cos(Th1)*sin(Th4) + 0.00062*sin(Th2 + Th3)*cos(Th4)*sin(Th1) + 0.00002*cos(Th1)*cos(Th4)*cos(Th5) - 0.00152*cos(Th1)*cos(Th4)*sin(Th5) - 0.00002*sin(Th2 + Th3)*cos(Th5)*sin(Th1)*sin(Th4) + 0.00152*sin(Th2 + Th3)*sin(Th1)*sin(Th4)*sin(Th5)) - 0.00004*sin(Th5) - 1.0*(0.05206*cos(Th2 + Th3)*cos(Th1)*cos(Th5) + 0.05206*sin(Th1)*sin(Th4)*sin(Th5) + 0.00023*cos(Th2 + Th3)*cos(Th1)*cos(Th6)*sin(Th5) - 0.05206*sin(Th2 + Th3)*cos(Th1)*cos(Th4)*sin(Th5) - 0.00023*cos(Th5)*cos(Th6)*sin(Th1)*sin(Th4) + 0.00023*sin(Th2 + Th3)*cos(Th1)*cos(Th4)*cos(Th5)*cos(Th6))*(0.02603*cos(Th4)*sin(Th1)*sin(Th5) + 0.000115*sin(Th1)*sin(Th4)*sin(Th6) - 0.000115*sin(Th2 + Th3)*cos(Th1)*cos(Th4)*sin(Th6) + 0.02603*sin(Th2 + Th3)*cos(Th1)*sin(Th4)*sin(Th5) - 0.000115*cos(Th4)*cos(Th5)*cos(Th6)*sin(Th1) - 0.000115*sin(Th2 + Th3)*cos(Th1)*cos(Th5)*cos(Th6)*sin(Th4)) - 4.0e-6*sin(Th5)*sin(Th6) + (0.02603*cos(Th2 + Th3)*cos(Th5)*sin(Th1) - 0.02603*cos(Th1)*sin(Th4)*sin(Th5) + 0.000115*cos(Th2 + Th3)*cos(Th6)*sin(Th1)*sin(Th5) - 0.02603*sin(Th2 + Th3)*cos(Th4)*sin(Th1)*sin(Th5) + 0.000115*cos(Th1)*cos(Th5)*cos(Th6)*sin(Th4) + 0.000115*sin(Th2 + Th3)*cos(Th4)*cos(Th5)*cos(Th6)*sin(Th1))*(0.05206*cos(Th1)*cos(Th4)*sin(Th5) + 0.00023*cos(Th1)*sin(Th4)*sin(Th6) + 0.00023*sin(Th2 + Th3)*cos(Th4)*sin(Th1)*sin(Th6) - 0.05206*sin(Th2 + Th3)*sin(Th1)*sin(Th4)*sin(Th5) - 0.00023*cos(Th1)*cos(Th4)*cos(Th5)*cos(Th6) + 0.00023*sin(Th2 + Th3)*cos(Th5)*cos(Th6)*sin(Th1)*sin(Th4)) + cos(Th2 + Th3)*(0.00062*cos(Th4) - 0.00002*cos(Th5)*sin(Th4) + 0.00152*sin(Th4)*sin(Th5))*(0.00152*sin(Th2 + Th3)*cos(Th5) + 0.00002*sin(Th2 + Th3)*sin(Th5) - 0.00002*cos(Th2 + Th3)*cos(Th4)*cos(Th5) + 0.00152*cos(Th2 + Th3)*cos(Th4)*sin(Th5)) - 0.5*cos(Th2 + Th3)*(0.00023*cos(Th4)*sin(Th6) - 0.05206*sin(Th4)*sin(Th5) + 0.00023*cos(Th5)*cos(Th6)*sin(Th4))*(0.05206*sin(Th2 + Th3)*cos(Th5) + 0.05206*cos(Th2 + Th3)*cos(Th4)*sin(Th5) + 0.00023*sin(Th2 + Th3)*cos(Th6)*sin(Th5) - 0.00023*cos(Th2 + Th3)*cos(Th4)*cos(Th5)*cos(Th6)) - 3.0e-6*cos(Th5)*cos(Th6)*sin(Th6))*dTh5*dTh5;
V456=(3.0e-6*sin(Th5) - 0.5*(0.000115*cos(Th6)*sin(Th1)*sin(Th4) - 0.000115*sin(Th2 + Th3)*cos(Th1)*cos(Th4)*cos(Th6) + 0.000115*cos(Th4)*cos(Th5)*sin(Th1)*sin(Th6) + 0.000115*sin(Th2 + Th3)*cos(Th1)*cos(Th5)*sin(Th4)*sin(Th6))*(0.05206*cos(Th2 + Th3)*cos(Th1)*sin(Th5) - 0.05206*cos(Th5)*sin(Th1)*sin(Th4) + 0.05206*sin(Th2 + Th3)*cos(Th1)*cos(Th4)*cos(Th5) - 0.00023*cos(Th6)*sin(Th1)*sin(Th4)*sin(Th5) - 0.00023*cos(Th2 + Th3)*cos(Th1)*cos(Th5)*cos(Th6) + 0.00023*sin(Th2 + Th3)*cos(Th1)*cos(Th4)*cos(Th6)*sin(Th5)) - 6.0e-6*cos(Th6)^2*sin(Th5) + 4.0e-6*cos(Th5)*cos(Th6) + 0.5*(0.000115*cos(Th1)*cos(Th6)*sin(Th4) + 0.000115*sin(Th2 + Th3)*cos(Th4)*cos(Th6)*sin(Th1) + 0.000115*cos(Th1)*cos(Th4)*cos(Th5)*sin(Th6) - 0.000115*sin(Th2 + Th3)*cos(Th5)*sin(Th1)*sin(Th4)*sin(Th6))*(0.05206*cos(Th2 + Th3)*sin(Th1)*sin(Th5) + 0.05206*cos(Th1)*cos(Th5)*sin(Th4) - 0.00023*cos(Th2 + Th3)*cos(Th5)*cos(Th6)*sin(Th1) + 0.05206*sin(Th2 + Th3)*cos(Th4)*cos(Th5)*sin(Th1) + 0.00023*cos(Th1)*cos(Th6)*sin(Th4)*sin(Th5) + 0.00023*sin(Th2 + Th3)*cos(Th4)*cos(Th6)*sin(Th1)*sin(Th5)) - 0.5*(0.05206*cos(Th5) + 0.00023*cos(Th6)*sin(Th5))*(0.5*cos(Th1)*cos(Th4) - 0.5*sin(Th2 + Th3)*sin(Th1)*sin(Th4))*(0.00023*sin(Th2 + Th3)*cos(Th6)*sin(Th1)*sin(Th4) - 0.00023*cos(Th1)*cos(Th4)*cos(Th6) + 0.00023*cos(Th2 + Th3)*sin(Th1)*sin(Th5)*sin(Th6) + 0.00023*cos(Th1)*cos(Th5)*sin(Th4)*sin(Th6) + 0.00023*sin(Th2 + Th3)*cos(Th4)*cos(Th5)*sin(Th1)*sin(Th6)) + 0.25*cos(Th2 + Th3)*(0.00023*cos(Th4)*cos(Th6) - 0.00023*cos(Th5)*sin(Th4)*sin(Th6))*(0.05206*cos(Th2 + Th3)*cos(Th4)*cos(Th5) - 0.05206*sin(Th2 + Th3)*sin(Th5) + 0.00023*sin(Th2 + Th3)*cos(Th5)*cos(Th6) + 0.00023*cos(Th2 + Th3)*cos(Th4)*cos(Th6)*sin(Th5)) - 0.000115*sin(Th6)*(cos(Th2 + Th3)*cos(Th1)*cos(Th5) + sin(Th1)*sin(Th4)*sin(Th5) - 1.0*sin(Th2 + Th3)*cos(Th1)*cos(Th4)*sin(Th5))*(0.05206*cos(Th4)*sin(Th1)*sin(Th5) + 0.00023*sin(Th1)*sin(Th4)*sin(Th6) - 0.00023*sin(Th2 + Th3)*cos(Th1)*cos(Th4)*sin(Th6) + 0.05206*sin(Th2 + Th3)*cos(Th1)*sin(Th4)*sin(Th5) - 0.00023*cos(Th4)*cos(Th5)*cos(Th6)*sin(Th1) - 0.00023*sin(Th2 + Th3)*cos(Th1)*cos(Th5)*cos(Th6)*sin(Th4)) - 0.000115*sin(Th6)*(cos(Th1)*sin(Th4)*sin(Th5) - 1.0*cos(Th2 + Th3)*cos(Th5)*sin(Th1) + sin(Th2 + Th3)*cos(Th4)*sin(Th1)*sin(Th5))*(0.05206*cos(Th1)*cos(Th4)*sin(Th5) + 0.00023*cos(Th1)*sin(Th4)*sin(Th6) + 0.00023*sin(Th2 + Th3)*cos(Th4)*sin(Th1)*sin(Th6) - 0.05206*sin(Th2 + Th3)*sin(Th1)*sin(Th4)*sin(Th5) - 0.00023*cos(Th1)*cos(Th4)*cos(Th5)*cos(Th6) + 0.00023*sin(Th2 + Th3)*cos(Th5)*cos(Th6)*sin(Th1)*sin(Th4)) + 0.5*(0.05206*cos(Th5) + 0.00023*cos(Th6)*sin(Th5))*(cos(Th4)*sin(Th1) + sin(Th2 + Th3)*cos(Th1)*sin(Th4))*(0.000115*cos(Th4)*cos(Th6)*sin(Th1) + 0.000115*sin(Th2 + Th3)*cos(Th1)*cos(Th6)*sin(Th4) + 0.000115*cos(Th2 + Th3)*cos(Th1)*sin(Th5)*sin(Th6) - 0.000115*cos(Th5)*sin(Th1)*sin(Th4)*sin(Th6) + 0.000115*sin(Th2 + Th3)*cos(Th1)*cos(Th4)*cos(Th5)*sin(Th6)) - 0.000115*cos(Th2 + Th3)*sin(Th6)*(sin(Th2 + Th3)*cos(Th5) + cos(Th2 + Th3)*cos(Th4)*sin(Th5))*(0.00023*cos(Th4)*sin(Th6) - 0.05206*sin(Th4)*sin(Th5) + 0.00023*cos(Th5)*cos(Th6)*sin(Th4)) + 0.25*cos(Th2 + Th3)*sin(Th4)*(0.05206*cos(Th5) + 0.00023*cos(Th6)*sin(Th5))*(0.00023*cos(Th2 + Th3)*cos(Th6)*sin(Th4) - 0.00023*sin(Th2 + Th3)*sin(Th5)*sin(Th6) + 0.00023*cos(Th2 + Th3)*cos(Th4)*cos(Th5)*sin(Th6)))*dTh5*dTh6;
%---------------------------
V461=(4.025e-6*cos(Th6)*sin(Th4) + 4.025e-6*cos(Th4)*cos(Th5)*sin(Th6) - 0.0000207*cos(Th6)*sin(Th2)*sin(Th4) + 4.9934e-6*cos(Th2)*cos(Th3)*cos(Th4)*sin(Th6) + 0.00002185*cos(Th2)*cos(Th3)*cos(Th6)*sin(Th4) + 0.000058013*cos(Th2)*cos(Th3)*sin(Th4)*sin(Th5) - 0.0000207*cos(Th4)*cos(Th5)*sin(Th2)*sin(Th6) - 4.9934e-6*cos(Th4)*sin(Th2)*sin(Th3)*sin(Th6) - 0.00002185*cos(Th6)*sin(Th2)*sin(Th3)*sin(Th4) - 0.000058013*sin(Th2)*sin(Th3)*sin(Th4)*sin(Th5) + 0.00002185*cos(Th2)*cos(Th3)*cos(Th4)*cos(Th5)*sin(Th6) + 4.9934e-6*cos(Th2)*cos(Th3)*cos(Th5)*cos(Th6)*sin(Th4) - 0.00002185*cos(Th4)*cos(Th5)*sin(Th2)*sin(Th3)*sin(Th6) - 4.9934e-6*cos(Th5)*cos(Th6)*sin(Th2)*sin(Th3)*sin(Th4))*dTh6*dTh1;
V462=(4.9934e-6*sin(Th4)*sin(Th6) - 0.000058013*cos(Th4)*sin(Th5) - 0.00002185*cos(Th4)*cos(Th6) - 4.9934e-6*cos(Th4)*cos(Th5)*cos(Th6) - 0.0000207*cos(Th4)*cos(Th6)*sin(Th3) + 0.00002185*cos(Th5)*sin(Th4)*sin(Th6) + 0.0000207*cos(Th5)*sin(Th3)*sin(Th4)*sin(Th6))*dTh6*dTh2;
V463=(4.9934e-6*sin(Th4)*sin(Th6) - 0.000058013*cos(Th4)*sin(Th5) - 0.00002185*cos(Th4)*cos(Th6) - 4.9934e-6*cos(Th4)*cos(Th5)*cos(Th6) - 0.5*cos(Th1)*(0.00023*cos(Th2 + Th3)*cos(Th6)*sin(Th4) - 0.00023*sin(Th2 + Th3)*sin(Th5)*sin(Th6) + 0.00023*cos(Th2 + Th3)*cos(Th4)*cos(Th5)*sin(Th6))*(0.05206*cos(Th4)*sin(Th1)*sin(Th5) + 0.00023*sin(Th1)*sin(Th4)*sin(Th6) - 0.00023*sin(Th2 + Th3)*cos(Th1)*cos(Th4)*sin(Th6) + 0.05206*sin(Th2 + Th3)*cos(Th1)*sin(Th4)*sin(Th5) - 0.00023*cos(Th4)*cos(Th5)*cos(Th6)*sin(Th1) - 0.00023*sin(Th2 + Th3)*cos(Th1)*cos(Th5)*cos(Th6)*sin(Th4)) + 0.00002185*cos(Th5)*sin(Th4)*sin(Th6) - 0.5*cos(Th2 + Th3)*(0.00023*cos(Th4)*sin(Th6) - 0.05206*sin(Th4)*sin(Th5) + 0.00023*cos(Th5)*cos(Th6)*sin(Th4))*(0.00023*sin(Th2 + Th3)*cos(Th6)*sin(Th4) + 0.00023*cos(Th2 + Th3)*sin(Th5)*sin(Th6) + 0.00023*sin(Th2 + Th3)*cos(Th4)*cos(Th5)*sin(Th6)) + 0.5*sin(Th1)*(0.00023*cos(Th2 + Th3)*cos(Th6)*sin(Th4) - 0.00023*sin(Th2 + Th3)*sin(Th5)*sin(Th6) + 0.00023*cos(Th2 + Th3)*cos(Th4)*cos(Th5)*sin(Th6))*(0.05206*cos(Th1)*cos(Th4)*sin(Th5) + 0.00023*cos(Th1)*sin(Th4)*sin(Th6) + 0.00023*sin(Th2 + Th3)*cos(Th4)*sin(Th1)*sin(Th6) - 0.05206*sin(Th2 + Th3)*sin(Th1)*sin(Th4)*sin(Th5) - 0.00023*cos(Th1)*cos(Th4)*cos(Th5)*cos(Th6) + 0.00023*sin(Th2 + Th3)*cos(Th5)*cos(Th6)*sin(Th1)*sin(Th4)) - 0.5*sin(Th2 + Th3)*(0.00023*cos(Th4)*sin(Th6) - 0.05206*sin(Th4)*sin(Th5) + 0.00023*cos(Th5)*cos(Th6)*sin(Th4))*(0.00023*cos(Th2 + Th3)*cos(Th6)*sin(Th4) - 0.00023*sin(Th2 + Th3)*sin(Th5)*sin(Th6) + 0.00023*cos(Th2 + Th3)*cos(Th4)*cos(Th5)*sin(Th6)) + 0.5*cos(Th2 + Th3)*cos(Th1)*(0.00023*cos(Th4)*sin(Th6) - 0.05206*sin(Th4)*sin(Th5) + 0.00023*cos(Th5)*cos(Th6)*sin(Th4))*(0.00023*cos(Th4)*cos(Th6)*sin(Th1) + 0.00023*sin(Th2 + Th3)*cos(Th1)*cos(Th6)*sin(Th4) + 0.00023*cos(Th2 + Th3)*cos(Th1)*sin(Th5)*sin(Th6) - 0.00023*cos(Th5)*sin(Th1)*sin(Th4)*sin(Th6) + 0.00023*sin(Th2 + Th3)*cos(Th1)*cos(Th4)*cos(Th5)*sin(Th6)) + 0.5*cos(Th2 + Th3)*sin(Th1)*(0.00023*cos(Th4)*sin(Th6) - 0.05206*sin(Th4)*sin(Th5) + 0.00023*cos(Th5)*cos(Th6)*sin(Th4))*(0.00023*sin(Th2 + Th3)*cos(Th6)*sin(Th1)*sin(Th4) - 0.00023*cos(Th1)*cos(Th4)*cos(Th6) + 0.00023*cos(Th2 + Th3)*sin(Th1)*sin(Th5)*sin(Th6) + 0.00023*cos(Th1)*cos(Th5)*sin(Th4)*sin(Th6) + 0.00023*sin(Th2 + Th3)*cos(Th4)*cos(Th5)*sin(Th1)*sin(Th6)))*dTh6*dTh3;
V464=(0.5*(0.000115*sin(Th2 + Th3)*cos(Th6)*sin(Th1)*sin(Th4) - 0.000115*cos(Th1)*cos(Th4)*cos(Th6) + 0.000115*cos(Th2 + Th3)*sin(Th1)*sin(Th5)*sin(Th6) + 0.000115*cos(Th1)*cos(Th5)*sin(Th4)*sin(Th6) + 0.000115*sin(Th2 + Th3)*cos(Th4)*cos(Th5)*sin(Th1)*sin(Th6))*(0.00023*cos(Th1)*cos(Th4)*sin(Th6) - 0.05206*cos(Th1)*sin(Th4)*sin(Th5) - 0.05206*sin(Th2 + Th3)*cos(Th4)*sin(Th1)*sin(Th5) - 0.00023*sin(Th2 + Th3)*sin(Th1)*sin(Th4)*sin(Th6) + 0.00023*cos(Th1)*cos(Th5)*cos(Th6)*sin(Th4) + 0.00023*sin(Th2 + Th3)*cos(Th4)*cos(Th5)*cos(Th6)*sin(Th1)) - 0.5*(0.000115*cos(Th4)*cos(Th6)*sin(Th1) + 0.000115*sin(Th2 + Th3)*cos(Th1)*cos(Th6)*sin(Th4) + 0.000115*cos(Th2 + Th3)*cos(Th1)*sin(Th5)*sin(Th6) - 0.000115*cos(Th5)*sin(Th1)*sin(Th4)*sin(Th6) + 0.000115*sin(Th2 + Th3)*cos(Th1)*cos(Th4)*cos(Th5)*sin(Th6))*(0.00023*cos(Th4)*sin(Th1)*sin(Th6) - 0.05206*sin(Th1)*sin(Th4)*sin(Th5) + 0.05206*sin(Th2 + Th3)*cos(Th1)*cos(Th4)*sin(Th5) + 0.00023*sin(Th2 + Th3)*cos(Th1)*sin(Th4)*sin(Th6) + 0.00023*cos(Th5)*cos(Th6)*sin(Th1)*sin(Th4) - 0.00023*sin(Th2 + Th3)*cos(Th1)*cos(Th4)*cos(Th5)*cos(Th6)) + 0.5*(0.000115*cos(Th6)*sin(Th1)*sin(Th4) - 0.000115*sin(Th2 + Th3)*cos(Th1)*cos(Th4)*cos(Th6) + 0.000115*cos(Th4)*cos(Th5)*sin(Th1)*sin(Th6) + 0.000115*sin(Th2 + Th3)*cos(Th1)*cos(Th5)*sin(Th4)*sin(Th6))*(0.05206*cos(Th4)*sin(Th1)*sin(Th5) + 0.00023*sin(Th1)*sin(Th4)*sin(Th6) - 0.00023*sin(Th2 + Th3)*cos(Th1)*cos(Th4)*sin(Th6) + 0.05206*sin(Th2 + Th3)*cos(Th1)*sin(Th4)*sin(Th5) - 0.00023*cos(Th4)*cos(Th5)*cos(Th6)*sin(Th1) - 0.00023*sin(Th2 + Th3)*cos(Th1)*cos(Th5)*cos(Th6)*sin(Th4)) + 0.5*(0.000115*cos(Th1)*cos(Th6)*sin(Th4) + 0.000115*sin(Th2 + Th3)*cos(Th4)*cos(Th6)*sin(Th1) + 0.000115*cos(Th1)*cos(Th4)*cos(Th5)*sin(Th6) - 0.000115*sin(Th2 + Th3)*cos(Th5)*sin(Th1)*sin(Th4)*sin(Th6))*(0.05206*cos(Th1)*cos(Th4)*sin(Th5) + 0.00023*cos(Th1)*sin(Th4)*sin(Th6) + 0.00023*sin(Th2 + Th3)*cos(Th4)*sin(Th1)*sin(Th6) - 0.05206*sin(Th2 + Th3)*sin(Th1)*sin(Th4)*sin(Th5) - 0.00023*cos(Th1)*cos(Th4)*cos(Th5)*cos(Th6) + 0.00023*sin(Th2 + Th3)*cos(Th5)*cos(Th6)*sin(Th1)*sin(Th4)) + 0.25*cos(Th2 + Th3)^2*(0.00023*cos(Th4)*cos(Th6) - 0.00023*cos(Th5)*sin(Th4)*sin(Th6))*(0.00023*cos(Th4)*sin(Th6) - 0.05206*sin(Th4)*sin(Th5) + 0.00023*cos(Th5)*cos(Th6)*sin(Th4)) - 0.25*cos(Th2 + Th3)*(0.05206*cos(Th4)*sin(Th5) + 0.00023*sin(Th4)*sin(Th6) - 0.00023*cos(Th4)*cos(Th5)*cos(Th6))*(0.00023*cos(Th2 + Th3)*cos(Th6)*sin(Th4) - 0.00023*sin(Th2 + Th3)*sin(Th5)*sin(Th6) + 0.00023*cos(Th2 + Th3)*cos(Th4)*cos(Th5)*sin(Th6)))*dTh6*dTh4;
V465=(0.5*(0.000115*cos(Th6)*sin(Th1)*sin(Th4) - 0.000115*sin(Th2 + Th3)*cos(Th1)*cos(Th4)*cos(Th6) + 0.000115*cos(Th4)*cos(Th5)*sin(Th1)*sin(Th6) + 0.000115*sin(Th2 + Th3)*cos(Th1)*cos(Th5)*sin(Th4)*sin(Th6))*(0.05206*cos(Th2 + Th3)*cos(Th1)*sin(Th5) - 0.05206*cos(Th5)*sin(Th1)*sin(Th4) + 0.05206*sin(Th2 + Th3)*cos(Th1)*cos(Th4)*cos(Th5) - 0.00023*cos(Th6)*sin(Th1)*sin(Th4)*sin(Th5) - 0.00023*cos(Th2 + Th3)*cos(Th1)*cos(Th5)*cos(Th6) + 0.00023*sin(Th2 + Th3)*cos(Th1)*cos(Th4)*cos(Th6)*sin(Th5)) - 0.000116*sin(Th5) - 4.0e-6*cos(Th5)*cos(Th6) - 0.5*(0.000115*cos(Th1)*cos(Th6)*sin(Th4) + 0.000115*sin(Th2 + Th3)*cos(Th4)*cos(Th6)*sin(Th1) + 0.000115*cos(Th1)*cos(Th4)*cos(Th5)*sin(Th6) - 0.000115*sin(Th2 + Th3)*cos(Th5)*sin(Th1)*sin(Th4)*sin(Th6))*(0.05206*cos(Th2 + Th3)*sin(Th1)*sin(Th5) + 0.05206*cos(Th1)*cos(Th5)*sin(Th4) - 0.00023*cos(Th2 + Th3)*cos(Th5)*cos(Th6)*sin(Th1) + 0.05206*sin(Th2 + Th3)*cos(Th4)*cos(Th5)*sin(Th1) + 0.00023*cos(Th1)*cos(Th6)*sin(Th4)*sin(Th5) + 0.00023*sin(Th2 + Th3)*cos(Th4)*cos(Th6)*sin(Th1)*sin(Th5)) + 0.5*(0.05206*cos(Th5) + 0.00023*cos(Th6)*sin(Th5))*(0.5*cos(Th1)*cos(Th4) - 0.5*sin(Th2 + Th3)*sin(Th1)*sin(Th4))*(0.00023*sin(Th2 + Th3)*cos(Th6)*sin(Th1)*sin(Th4) - 0.00023*cos(Th1)*cos(Th4)*cos(Th6) + 0.00023*cos(Th2 + Th3)*sin(Th1)*sin(Th5)*sin(Th6) + 0.00023*cos(Th1)*cos(Th5)*sin(Th4)*sin(Th6) + 0.00023*sin(Th2 + Th3)*cos(Th4)*cos(Th5)*sin(Th1)*sin(Th6)) - 0.25*cos(Th2 + Th3)*(0.00023*cos(Th4)*cos(Th6) - 0.00023*cos(Th5)*sin(Th4)*sin(Th6))*(0.05206*cos(Th2 + Th3)*cos(Th4)*cos(Th5) - 0.05206*sin(Th2 + Th3)*sin(Th5) + 0.00023*sin(Th2 + Th3)*cos(Th5)*cos(Th6) + 0.00023*cos(Th2 + Th3)*cos(Th4)*cos(Th6)*sin(Th5)) - 0.000115*sin(Th6)*(cos(Th2 + Th3)*cos(Th1)*cos(Th5) + sin(Th1)*sin(Th4)*sin(Th5) - 1.0*sin(Th2 + Th3)*cos(Th1)*cos(Th4)*sin(Th5))*(0.05206*cos(Th4)*sin(Th1)*sin(Th5) + 0.00023*sin(Th1)*sin(Th4)*sin(Th6) - 0.00023*sin(Th2 + Th3)*cos(Th1)*cos(Th4)*sin(Th6) + 0.05206*sin(Th2 + Th3)*cos(Th1)*sin(Th4)*sin(Th5) - 0.00023*cos(Th4)*cos(Th5)*cos(Th6)*sin(Th1) - 0.00023*sin(Th2 + Th3)*cos(Th1)*cos(Th5)*cos(Th6)*sin(Th4)) - 0.000115*sin(Th6)*(cos(Th1)*sin(Th4)*sin(Th5) - 1.0*cos(Th2 + Th3)*cos(Th5)*sin(Th1) + sin(Th2 + Th3)*cos(Th4)*sin(Th1)*sin(Th5))*(0.05206*cos(Th1)*cos(Th4)*sin(Th5) + 0.00023*cos(Th1)*sin(Th4)*sin(Th6) + 0.00023*sin(Th2 + Th3)*cos(Th4)*sin(Th1)*sin(Th6) - 0.05206*sin(Th2 + Th3)*sin(Th1)*sin(Th4)*sin(Th5) - 0.00023*cos(Th1)*cos(Th4)*cos(Th5)*cos(Th6) + 0.00023*sin(Th2 + Th3)*cos(Th5)*cos(Th6)*sin(Th1)*sin(Th4)) - 0.5*(0.05206*cos(Th5) + 0.00023*cos(Th6)*sin(Th5))*(cos(Th4)*sin(Th1) + sin(Th2 + Th3)*cos(Th1)*sin(Th4))*(0.000115*cos(Th4)*cos(Th6)*sin(Th1) + 0.000115*sin(Th2 + Th3)*cos(Th1)*cos(Th6)*sin(Th4) + 0.000115*cos(Th2 + Th3)*cos(Th1)*sin(Th5)*sin(Th6) - 0.000115*cos(Th5)*sin(Th1)*sin(Th4)*sin(Th6) + 0.000115*sin(Th2 + Th3)*cos(Th1)*cos(Th4)*cos(Th5)*sin(Th6)) - 0.000115*cos(Th2 + Th3)*sin(Th6)*(sin(Th2 + Th3)*cos(Th5) + cos(Th2 + Th3)*cos(Th4)*sin(Th5))*(0.00023*cos(Th4)*sin(Th6) - 0.05206*sin(Th4)*sin(Th5) + 0.00023*cos(Th5)*cos(Th6)*sin(Th4)) - 0.25*cos(Th2 + Th3)*sin(Th4)*(0.05206*cos(Th5) + 0.00023*cos(Th6)*sin(Th5))*(0.00023*cos(Th2 + Th3)*cos(Th6)*sin(Th4) - 0.00023*sin(Th2 + Th3)*sin(Th5)*sin(Th6) + 0.00023*cos(Th2 + Th3)*cos(Th4)*cos(Th5)*sin(Th6)))*dTh6*dTh5;
V466=((0.5*(cos(Th2 + Th3)*cos(Th1)*cos(Th5) + sin(Th1)*sin(Th4)*sin(Th5) - 1.0*sin(Th2 + Th3)*cos(Th1)*cos(Th4)*sin(Th5))*(0.00023*cos(Th2 + Th3)*cos(Th6)*sin(Th4) - 0.00023*sin(Th2 + Th3)*sin(Th5)*sin(Th6) + 0.00023*cos(Th2 + Th3)*cos(Th4)*cos(Th5)*sin(Th6)) + 0.5*(0.00023*sin(Th6)*(cos(Th2 + Th3)*cos(Th1)*sin(Th5) - 1.0*cos(Th5)*sin(Th1)*sin(Th4) + sin(Th2 + Th3)*cos(Th1)*cos(Th4)*cos(Th5)) + 0.00023*cos(Th6)*(cos(Th4)*sin(Th1) + sin(Th2 + Th3)*cos(Th1)*sin(Th4)))*(sin(Th2 + Th3)*cos(Th5) + cos(Th2 + Th3)*cos(Th4)*sin(Th5)))*(0.05206*cos(Th1)*cos(Th4)*sin(Th5) + 0.00023*cos(Th1)*sin(Th4)*sin(Th6) + 0.00023*sin(Th2 + Th3)*cos(Th4)*sin(Th1)*sin(Th6) - 0.05206*sin(Th2 + Th3)*sin(Th1)*sin(Th4)*sin(Th5) - 0.00023*cos(Th1)*cos(Th4)*cos(Th5)*cos(Th6) + 0.00023*sin(Th2 + Th3)*cos(Th5)*cos(Th6)*sin(Th1)*sin(Th4)) - (0.5*(cos(Th1)*sin(Th4)*sin(Th5) - 1.0*cos(Th2 + Th3)*cos(Th5)*sin(Th1) + sin(Th2 + Th3)*cos(Th4)*sin(Th1)*sin(Th5))*(0.00023*cos(Th2 + Th3)*cos(Th6)*sin(Th4) - 0.00023*sin(Th2 + Th3)*sin(Th5)*sin(Th6) + 0.00023*cos(Th2 + Th3)*cos(Th4)*cos(Th5)*sin(Th6)) + 0.5*(sin(Th2 + Th3)*cos(Th5) + cos(Th2 + Th3)*cos(Th4)*sin(Th5))*(0.00023*cos(Th6)*(cos(Th1)*cos(Th4) - 1.0*sin(Th2 + Th3)*sin(Th1)*sin(Th4)) - 0.00023*sin(Th6)*(cos(Th2 + Th3)*sin(Th1)*sin(Th5) + cos(Th1)*cos(Th5)*sin(Th4) + sin(Th2 + Th3)*cos(Th4)*cos(Th5)*sin(Th1))))*(0.05206*cos(Th4)*sin(Th1)*sin(Th5) + 0.00023*sin(Th1)*sin(Th4)*sin(Th6) - 0.00023*sin(Th2 + Th3)*cos(Th1)*cos(Th4)*sin(Th6) + 0.05206*sin(Th2 + Th3)*cos(Th1)*sin(Th4)*sin(Th5) - 0.00023*cos(Th4)*cos(Th5)*cos(Th6)*sin(Th1) - 0.00023*sin(Th2 + Th3)*cos(Th1)*cos(Th5)*cos(Th6)*sin(Th4)) + 4.0e-6*sin(Th5)*sin(Th6) - 0.5*cos(Th2 + Th3)*(0.00023*cos(Th4)*sin(Th6) - 0.05206*sin(Th4)*sin(Th5) + 0.00023*cos(Th5)*cos(Th6)*sin(Th4))*(0.00023*cos(Th2 + Th3)*sin(Th4)*sin(Th6) + 0.00023*sin(Th2 + Th3)*cos(Th6)*sin(Th5) - 0.00023*cos(Th2 + Th3)*cos(Th4)*cos(Th5)*cos(Th6)))*dTh6*dTh6;
%---------------------------
V4 = V411+V412+V413+V414+V415+V416+V421+V422+V423+V424+V425+V426+...
     V431+V432+V433+V434+V435+V436+V441+V442+V443+V444+V445+V446+...
     V451+V452+V453+V454+V455+V456+V461+V462+V463+V464+V465+V466;
end
